simulink model "c00013M_harness"  (R2018a)
settings: Solver=FixedStepAuto  StartTime=0.0  StopTime=300  FixedStep=0.1  RelTol=1e-3
undefined symbols (not defined in the file): A1, hmax, PriorityTank, R1, R2, sigbuilder_block, TempThreshold
(part 1 of 93)
settings Model: Creator=aarrieta  LastModifiedBy=umarkiegi

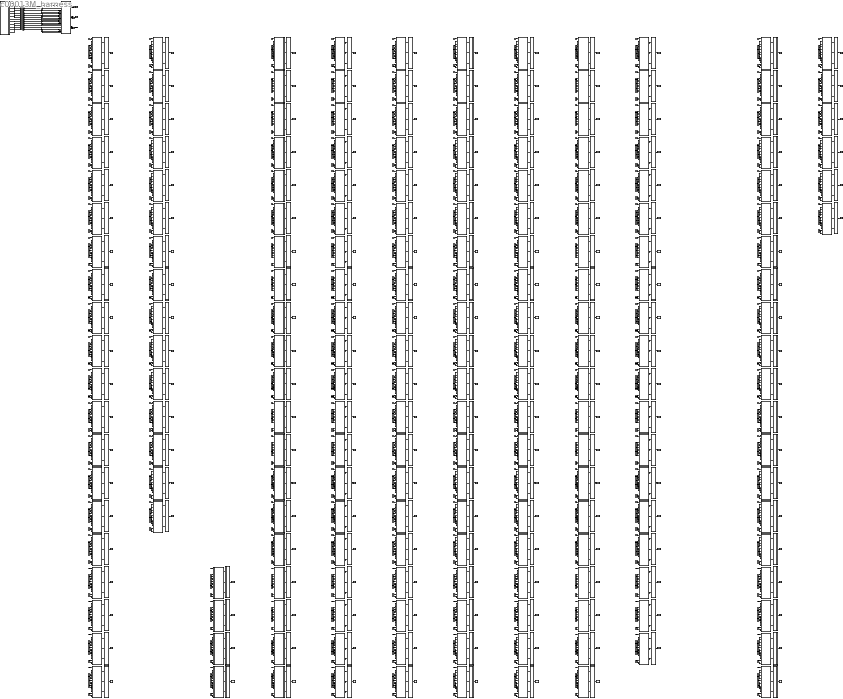
== system c00013M_harness ==
  CPSUT : Subsystem
  Eval : Subsystem
  Eval1 : Subsystem
  Eval10 : Subsystem
  Eval100 : Subsystem
  Eval101 : Subsystem
  Eval102 : Subsystem
  Eval103 : Subsystem
  Eval104 : Subsystem
  Eval105 : Subsystem
  Eval106 : Subsystem
  Eval107 : Subsystem
  Eval108 : Subsystem
  Eval109 : Subsystem
  Eval11 : Subsystem
  Eval110 : Subsystem
  Eval111 : Subsystem
  Eval112 : Subsystem
  Eval113 : Subsystem
  Eval114 : Subsystem
  Eval115 : Subsystem
  Eval116 : Subsystem
  Eval117 : Subsystem
  Eval118 : Subsystem
  Eval119 : Subsystem
  Eval12 : Subsystem
  Eval120 : Subsystem
  Eval121 : Subsystem
  Eval122 : Subsystem
  Eval123 : Subsystem
  Eval124 : Subsystem
  Eval125 : Subsystem
  Eval126 : Subsystem
  Eval127 : Subsystem
  Eval128 : Subsystem
  Eval129 : Subsystem
  Eval13 : Subsystem
  Eval130 : Subsystem
  Eval131 : Subsystem
  Eval132 : Subsystem
  Eval133 : Subsystem
  Eval134 : Subsystem
  Eval135 : Subsystem
  Eval136 : Subsystem
  Eval137 : Subsystem
  Eval138 : Subsystem
  Eval139 : Subsystem
  Eval14 : Subsystem
  Eval140 : Subsystem
  Eval141 : Subsystem
  Eval142 : Subsystem
  Eval143 : Subsystem
  Eval144 : Subsystem
  Eval145 : Subsystem
  Eval146 : Subsystem
  Eval147 : Subsystem
  Eval148 : Subsystem
  Eval149 : Subsystem
  Eval15 : Subsystem
  Eval150 : Subsystem
  Eval151 : Subsystem
  Eval152 : Subsystem
  Eval153 : Subsystem
  Eval154 : Subsystem
  Eval155 : Subsystem
  Eval156 : Subsystem
  Eval157 : Subsystem
  Eval158 : Subsystem
  Eval159 : Subsystem
  Eval16 : Subsystem
  Eval160 : Subsystem
  Eval161 : Subsystem
  Eval162 : Subsystem
  Eval163 : Subsystem
  Eval164 : Subsystem
  Eval165 : Subsystem
  Eval166 : Subsystem
  Eval167 : Subsystem
  Eval168 : Subsystem
  Eval169 : Subsystem
  Eval17 : Subsystem
  Eval170 : Subsystem
  Eval171 : Subsystem
  Eval172 : Subsystem
  Eval173 : Subsystem
  Eval174 : Subsystem
  Eval175 : Subsystem
  Eval176 : Subsystem
  Eval177 : Subsystem
  Eval178 : Subsystem
  Eval179 : Subsystem
  Eval18 : Subsystem
  Eval180 : Subsystem
  Eval181 : Subsystem
  Eval182 : Subsystem
  Eval183 : Subsystem
  Eval184 : Subsystem
  Eval185 : Subsystem
  Eval186 : Subsystem
  Eval187 : Subsystem
  Eval188 : Subsystem
  Eval189 : Subsystem
  Eval19 : Subsystem
  Eval190 : Subsystem
  Eval191 : Subsystem
  Eval192 : Subsystem
  Eval193 : Subsystem
  Eval194 : Subsystem
  Eval195 : Subsystem
  Eval196 : Subsystem
  Eval197 : Subsystem
  Eval198 : Subsystem
  Eval2 : Subsystem
  Eval20 : Subsystem
  Eval21 : Subsystem
  Eval22 : Subsystem
  Eval220 : Subsystem
  Eval221 : Subsystem
  Eval222 : Subsystem
  Eval223 : Subsystem
  Eval224 : Subsystem
  Eval225 : Subsystem
  Eval226 : Subsystem
  Eval227 : Subsystem
  Eval228 : Subsystem
  Eval229 : Subsystem
  Eval23 : Subsystem
  Eval230 : Subsystem
  Eval231 : Subsystem
  Eval232 : Subsystem
  Eval233 : Subsystem
  Eval234 : Subsystem
  Eval235 : Subsystem
  Eval236 : Subsystem
  Eval237 : Subsystem
  Eval238 : Subsystem
  Eval239 : Subsystem
  Eval24 : Subsystem
  Eval240 : Subsystem
  Eval241 : Subsystem
  Eval242 : Subsystem
  Eval243 : Subsystem
  Eval244 : Subsystem
  Eval245 : Subsystem
  Eval25 : Subsystem
  Eval26 : Subsystem
  Eval27 : Subsystem
  Eval28 : Subsystem
  Eval29 : Subsystem
  Eval3 : Subsystem
  Eval30 : Subsystem
  Eval31 : Subsystem
  Eval32 : Subsystem
  Eval33 : Subsystem
  Eval34 : Subsystem
  Eval4 : Subsystem
  Eval5 : Subsystem
  Eval56 : Subsystem
  Eval57 : Subsystem
  Eval58 : Subsystem
  Eval59 : Subsystem
  Eval6 : Subsystem
  Eval60 : Subsystem
  Eval61 : Subsystem
  Eval62 : Subsystem
  Eval63 : Subsystem
  Eval64 : Subsystem
  Eval65 : Subsystem
  Eval66 : Subsystem
  Eval67 : Subsystem
  Eval68 : Subsystem
  Eval69 : Subsystem
  Eval7 : Subsystem
  Eval70 : Subsystem
  Eval71 : Subsystem
  Eval72 : Subsystem
  Eval73 : Subsystem
  Eval74 : Subsystem
  Eval75 : Subsystem
  Eval76 : Subsystem
  Eval77 : Subsystem
  Eval78 : Subsystem
  Eval79 : Subsystem
  Eval8 : Subsystem
  Eval80 : Subsystem
  Eval81 : Subsystem
  Eval82 : Subsystem
  Eval83 : Subsystem
  Eval84 : Subsystem
  Eval85 : Subsystem
  Eval86 : Subsystem
  Eval87 : Subsystem
  Eval88 : Subsystem
  Eval89 : Subsystem
  Eval9 : Subsystem
  Eval90 : Subsystem
  Eval91 : Subsystem
  Eval92 : Subsystem
  Eval93 : Subsystem
  Eval94 : Subsystem
  Eval95 : Subsystem
  Eval96 : Subsystem
  Eval97 : Subsystem
  Eval98 : Subsystem
  Eval99 : Subsystem
  Inputs : Subsystem  Tag=STV Subsys  LoadFcn=sigbuilder_block('load');  StartFcn=sigbuilder_block('start');  StopFcn=sigbuilder_block('stop');  ClipboardFcn=sigbuilder_block('clipboard');  mask(Sigbuilder block){tuvar=[0:10]}
      mask init:
      | if ~strcmp(get_param(bdroot(gcb),'SimulationStatus'),'stopped'),tuvar = sigbuilder_block('maskInit'); end
      settings: CopyFcn=sigbuilder_block('copy');  DeleteFcn=sigbuilder_block('delete');  ModelCloseFcn=sigbuilder_block('modelClose');  PreSaveFcn=sigbuilder_block('preSave');  PauseFcn=sigbuilder_block('pause');  ContinueFcn=sigbuilder_block('continue');  NameChangeFcn=sigbuilder_block('namechange');  OpenFcn=sigbuilder_block('open',[276.75 163.5 675.75 486.75 ]);  CloseFcn=sigbuilder_block('close');
      mask Display: plot(0, 0, 100, 100,[2, 2, 32, 32, 2], [68, 8, 8, 68, 68],[32, 2], [38, 38], [32, 19, 2],[53, 60, 44], [32, 17, 17, 2],[16, 16, 31, 31]);txt = getActiveGroup(gcbh);text(2, 100, txt,'verticalAlignment', 'top');
  M001 : Subsystem
  M002 : Subsystem
  M003 : Subsystem
  M004 : Subsystem
  M005 : Subsystem
  M006 : Subsystem
  M007 : Subsystem
  M008 : Subsystem
  M009 : Subsystem
  M010 : Subsystem
  M011 : Subsystem
  M012 : Subsystem
  M013 : Subsystem
  M014 : Subsystem
  M015 : Subsystem
  M016 : Subsystem
  M017 : Subsystem
  M018 : Subsystem
  M019 : Subsystem
  M020 : Subsystem
  M021 : Subsystem
  M022 : Subsystem
  M023 : Subsystem
  M024 : Subsystem
  M025 : Subsystem
  M026 : Subsystem
  M027 : Subsystem
  M028 : Subsystem
  M029 : Subsystem
  M030 : Subsystem
  M031 : Subsystem
  M032 : Subsystem
  M033 : Subsystem
  M034 : Subsystem
  M035 : Subsystem
  M057 : Subsystem
  M058 : Subsystem
  M059 : Subsystem
  M060 : Subsystem
  M061 : Subsystem
  M062 : Subsystem
  M063 : Subsystem
  M064 : Subsystem
  M065 : Subsystem
  M066 : Subsystem
  M067 : Subsystem
  M068 : Subsystem
  M069 : Subsystem
  M070 : Subsystem
  M071 : Subsystem
  M072 : Subsystem
  M073 : Subsystem
  M074 : Subsystem
  M075 : Subsystem
  M076 : Subsystem
  M077 : Subsystem
  M078 : Subsystem
  M079 : Subsystem
  M080 : Subsystem
  M081 : Subsystem
  M082 : Subsystem
  M083 : Subsystem
  M084 : Subsystem
  M085 : Subsystem
  M086 : Subsystem
  M087 : Subsystem
  M088 : Subsystem
  M089 : Subsystem
  M090 : Subsystem
  M091 : Subsystem
  M092 : Subsystem
  M093 : Subsystem
  M094 : Subsystem
  M095 : Subsystem
  M096 : Subsystem
  M097 : Subsystem
  M098 : Subsystem
  M099 : Subsystem
  M100 : Subsystem
  M101 : Subsystem
  M102 : Subsystem
  M103 : Subsystem
  M104 : Subsystem
  M105 : Subsystem
  M106 : Subsystem
  M107 : Subsystem
  M108 : Subsystem
  M109 : Subsystem
  M110 : Subsystem
  M111 : Subsystem
  M112 : Subsystem
  M113 : Subsystem
  M114 : Subsystem
  M115 : Subsystem
  M116 : Subsystem
  M117 : Subsystem
  M118 : Subsystem
  M119 : Subsystem
  M120 : Subsystem
  M121 : Subsystem
  M122 : Subsystem
  M123 : Subsystem
  M124 : Subsystem
  M125 : Subsystem
  M126 : Subsystem
  M127 : Subsystem
  M128 : Subsystem
  M129 : Subsystem
  M130 : Subsystem
  M131 : Subsystem
  M132 : Subsystem
  M133 : Subsystem
  M134 : Subsystem
  M135 : Subsystem
  M136 : Subsystem
  M137 : Subsystem
  M138 : Subsystem
  M139 : Subsystem
  M140 : Subsystem
  M141 : Subsystem
  M142 : Subsystem
  M143 : Subsystem
  M144 : Subsystem
  M145 : Subsystem
  M146 : Subsystem
  M147 : Subsystem
  M148 : Subsystem
  M149 : Subsystem
  M150 : Subsystem
  M151 : Subsystem
  M152 : Subsystem
  M153 : Subsystem
  M154 : Subsystem
  M155 : Subsystem
  M156 : Subsystem
  M157 : Subsystem
  M158 : Subsystem
  M159 : Subsystem
  M160 : Subsystem
  M161 : Subsystem
  M162 : Subsystem
  M163 : Subsystem
  M164 : Subsystem
  M165 : Subsystem
  M166 : Subsystem
  M167 : Subsystem
  M168 : Subsystem
  M169 : Subsystem
  M170 : Subsystem
  M171 : Subsystem
  M172 : Subsystem
  M173 : Subsystem
  M174 : Subsystem
  M175 : Subsystem
  M176 : Subsystem
  M177 : Subsystem
  M178 : Subsystem
  M179 : Subsystem
  M180 : Subsystem
  M181 : Subsystem
  M182 : Subsystem
  M183 : Subsystem
  M184 : Subsystem
  M185 : Subsystem
  M186 : Subsystem
  M187 : Subsystem
  M188 : Subsystem
  M189 : Subsystem
  M190 : Subsystem
  M191 : Subsystem
  M192 : Subsystem
  M193 : Subsystem
  M194 : Subsystem
  M195 : Subsystem
  M196 : Subsystem
  M197 : Subsystem
  M198 : Subsystem
  M199 : Subsystem
  M221 : Subsystem
  M222 : Subsystem
  M223 : Subsystem
  M224 : Subsystem
  M225 : Subsystem
  M226 : Subsystem
  M227 : Subsystem
  M228 : Subsystem
  M229 : Subsystem
  M230 : Subsystem
  M231 : Subsystem
  M232 : Subsystem
  M233 : Subsystem
  M234 : Subsystem
  M235 : Subsystem
  M236 : Subsystem
  M237 : Subsystem
  M238 : Subsystem
  M239 : Subsystem
  M240 : Subsystem
  M241 : Subsystem
  M242 : Subsystem
  M243 : Subsystem
  M244 : Subsystem
  M245 : Subsystem
  M246 : Subsystem
  To Workspace : ToWorkspace  VariableName=mutant001  SampleTime=-1
  To Workspace1 : ToWorkspace  VariableName=mutant002  SampleTime=-1
  To Workspace10 : ToWorkspace  VariableName=mutant011  SampleTime=-1
  To Workspace100 : ToWorkspace  VariableName=mutant101  SampleTime=-1
  To Workspace101 : ToWorkspace  VariableName=mutant102  SampleTime=-1
  To Workspace102 : ToWorkspace  VariableName=mutant103  SampleTime=-1
  To Workspace103 : ToWorkspace  VariableName=mutant104  SampleTime=-1
  To Workspace104 : ToWorkspace  VariableName=mutant105  SampleTime=-1
  To Workspace105 : ToWorkspace  VariableName=mutant106  SampleTime=-1
  To Workspace106 : ToWorkspace  VariableName=mutant107  SampleTime=-1
  To Workspace107 : ToWorkspace  VariableName=mutant108  SampleTime=-1
  To Workspace108 : ToWorkspace  VariableName=mutant109  SampleTime=-1
  To Workspace109 : ToWorkspace  VariableName=mutant110  SampleTime=-1
  To Workspace11 : ToWorkspace  VariableName=mutant012  SampleTime=-1
  To Workspace110 : ToWorkspace  VariableName=mutant111  SampleTime=-1
  To Workspace111 : ToWorkspace  VariableName=mutant112  SampleTime=-1
  To Workspace112 : ToWorkspace  VariableName=mutant113  SampleTime=-1
  To Workspace113 : ToWorkspace  VariableName=mutant114  SampleTime=-1
  To Workspace114 : ToWorkspace  VariableName=mutant115  SampleTime=-1
  To Workspace115 : ToWorkspace  VariableName=mutant116  SampleTime=-1
  To Workspace116 : ToWorkspace  VariableName=mutant117  SampleTime=-1
  To Workspace117 : ToWorkspace  VariableName=mutant118  SampleTime=-1
  To Workspace118 : ToWorkspace  VariableName=mutant119  SampleTime=-1
  To Workspace119 : ToWorkspace  VariableName=mutant120  SampleTime=-1
  To Workspace12 : ToWorkspace  VariableName=mutant013  SampleTime=-1
  To Workspace120 : ToWorkspace  VariableName=mutant121  SampleTime=-1
  To Workspace121 : ToWorkspace  VariableName=mutant122  SampleTime=-1
  To Workspace122 : ToWorkspace  VariableName=mutant123  SampleTime=-1
  To Workspace123 : ToWorkspace  VariableName=mutant124  SampleTime=-1
  To Workspace124 : ToWorkspace  VariableName=mutant125  SampleTime=-1
  To Workspace125 : ToWorkspace  VariableName=mutant126  SampleTime=-1
  To Workspace126 : ToWorkspace  VariableName=mutant127  SampleTime=-1
  To Workspace127 : ToWorkspace  VariableName=mutant128  SampleTime=-1
  To Workspace128 : ToWorkspace  VariableName=mutant129  SampleTime=-1
  To Workspace129 : ToWorkspace  VariableName=mutant130  SampleTime=-1
  To Workspace13 : ToWorkspace  VariableName=mutant014  SampleTime=-1
  To Workspace130 : ToWorkspace  VariableName=mutant131  SampleTime=-1
  To Workspace131 : ToWorkspace  VariableName=mutant132  SampleTime=-1
  To Workspace132 : ToWorkspace  VariableName=mutant133  SampleTime=-1
  To Workspace133 : ToWorkspace  VariableName=mutant134  SampleTime=-1
  To Workspace134 : ToWorkspace  VariableName=mutant135  SampleTime=-1
  To Workspace135 : ToWorkspace  VariableName=mutant136  SampleTime=-1
  To Workspace136 : ToWorkspace  VariableName=mutant137  SampleTime=-1
  To Workspace137 : ToWorkspace  VariableName=mutant138  SampleTime=-1
  To Workspace138 : ToWorkspace  VariableName=mutant139  SampleTime=-1
  To Workspace139 : ToWorkspace  VariableName=mutant140  SampleTime=-1
  To Workspace14 : ToWorkspace  VariableName=mutant015  SampleTime=-1
  To Workspace140 : ToWorkspace  VariableName=mutant141  SampleTime=-1
  To Workspace141 : ToWorkspace  VariableName=mutant142  SampleTime=-1
  To Workspace142 : ToWorkspace  VariableName=mutant143  SampleTime=-1
  To Workspace143 : ToWorkspace  VariableName=mutant144  SampleTime=-1
  To Workspace144 : ToWorkspace  VariableName=mutant145  SampleTime=-1
  To Workspace145 : ToWorkspace  VariableName=mutant146  SampleTime=-1
  To Workspace146 : ToWorkspace  VariableName=mutant147  SampleTime=-1
  To Workspace147 : ToWorkspace  VariableName=mutant148  SampleTime=-1
  To Workspace148 : ToWorkspace  VariableName=mutant149  SampleTime=-1
  To Workspace149 : ToWorkspace  VariableName=mutant150  SampleTime=-1
  To Workspace15 : ToWorkspace  VariableName=mutant016  SampleTime=-1
  To Workspace150 : ToWorkspace  VariableName=mutant151  SampleTime=-1
  To Workspace151 : ToWorkspace  VariableName=mutant152  SampleTime=-1
  To Workspace152 : ToWorkspace  VariableName=mutant153  SampleTime=-1
  To Workspace153 : ToWorkspace  VariableName=mutant154  SampleTime=-1
  To Workspace154 : ToWorkspace  VariableName=mutant155  SampleTime=-1
  To Workspace155 : ToWorkspace  VariableName=mutant156  SampleTime=-1
  To Workspace156 : ToWorkspace  VariableName=mutant157  SampleTime=-1
  To Workspace157 : ToWorkspace  VariableName=mutant158  SampleTime=-1
  To Workspace158 : ToWorkspace  VariableName=mutant159  SampleTime=-1
  To Workspace159 : ToWorkspace  VariableName=mutant160  SampleTime=-1
  To Workspace16 : ToWorkspace  VariableName=mutant017  SampleTime=-1
  To Workspace160 : ToWorkspace  VariableName=mutant161  SampleTime=-1
  To Workspace161 : ToWorkspace  VariableName=mutant162  SampleTime=-1
  To Workspace162 : ToWorkspace  VariableName=mutant163  SampleTime=-1
  To Workspace163 : ToWorkspace  VariableName=mutant164  SampleTime=-1
  To Workspace164 : ToWorkspace  VariableName=mutant165  SampleTime=-1
  To Workspace165 : ToWorkspace  VariableName=mutant166  SampleTime=-1
  To Workspace166 : ToWorkspace  VariableName=mutant167  SampleTime=-1
  To Workspace167 : ToWorkspace  VariableName=mutant168  SampleTime=-1
  To Workspace168 : ToWorkspace  VariableName=mutant169  SampleTime=-1
  To Workspace169 : ToWorkspace  VariableName=mutant170  SampleTime=-1
  To Workspace17 : ToWorkspace  VariableName=mutant018  SampleTime=-1
  To Workspace170 : ToWorkspace  VariableName=mutant171  SampleTime=-1
  To Workspace171 : ToWorkspace  VariableName=mutant172  SampleTime=-1
  To Workspace172 : ToWorkspace  VariableName=mutant173  SampleTime=-1
  To Workspace173 : ToWorkspace  VariableName=mutant174  SampleTime=-1
  To Workspace174 : ToWorkspace  VariableName=mutant175  SampleTime=-1
  To Workspace175 : ToWorkspace  VariableName=mutant176  SampleTime=-1
  To Workspace176 : ToWorkspace  VariableName=mutant177  SampleTime=-1
  To Workspace177 : ToWorkspace  VariableName=mutant178  SampleTime=-1
  To Workspace178 : ToWorkspace  VariableName=mutant179  SampleTime=-1
  To Workspace179 : ToWorkspace  VariableName=mutant180  SampleTime=-1
  To Workspace18 : ToWorkspace  VariableName=mutant019  SampleTime=-1
  To Workspace180 : ToWorkspace  VariableName=mutant181  SampleTime=-1
  To Workspace181 : ToWorkspace  VariableName=mutant182  SampleTime=-1
  To Workspace182 : ToWorkspace  VariableName=mutant183  SampleTime=-1
  To Workspace183 : ToWorkspace  VariableName=mutant184  SampleTime=-1
  To Workspace184 : ToWorkspace  VariableName=mutant185  SampleTime=-1
  To Workspace185 : ToWorkspace  VariableName=mutant186  SampleTime=-1
  To Workspace186 : ToWorkspace  VariableName=mutant187  SampleTime=-1
  To Workspace187 : ToWorkspace  VariableName=mutant188  SampleTime=-1
  To Workspace188 : ToWorkspace  VariableName=mutant189  SampleTime=-1
  To Workspace189 : ToWorkspace  VariableName=mutant190  SampleTime=-1
  To Workspace19 : ToWorkspace  VariableName=mutant020  SampleTime=-1
  To Workspace190 : ToWorkspace  VariableName=mutant191  SampleTime=-1
  To Workspace191 : ToWorkspace  VariableName=mutant192  SampleTime=-1
  To Workspace192 : ToWorkspace  VariableName=mutant193  SampleTime=-1
  To Workspace193 : ToWorkspace  VariableName=mutant194  SampleTime=-1
  To Workspace194 : ToWorkspace  VariableName=mutant195  SampleTime=-1
  To Workspace195 : ToWorkspace  VariableName=mutant196  SampleTime=-1
  To Workspace196 : ToWorkspace  VariableName=mutant197  SampleTime=-1
  To Workspace197 : ToWorkspace  VariableName=mutant198  SampleTime=-1
  To Workspace198 : ToWorkspace  VariableName=mutant199  SampleTime=-1
  To Workspace2 : ToWorkspace  VariableName=mutant003  SampleTime=-1
  To Workspace20 : ToWorkspace  VariableName=mutant021  SampleTime=-1
  To Workspace21 : ToWorkspace  VariableName=mutant022  SampleTime=-1
  To Workspace22 : ToWorkspace  VariableName=mutant023  SampleTime=-1
  To Workspace220 : ToWorkspace  VariableName=mutant221  SampleTime=-1
  To Workspace221 : ToWorkspace  VariableName=mutant222  SampleTime=-1
  To Workspace222 : ToWorkspace  VariableName=mutant223  SampleTime=-1
  To Workspace223 : ToWorkspace  VariableName=mutant224  SampleTime=-1
  To Workspace224 : ToWorkspace  VariableName=mutant225  SampleTime=-1
  To Workspace225 : ToWorkspace  VariableName=mutant226  SampleTime=-1
  To Workspace226 : ToWorkspace  VariableName=mutant227  SampleTime=-1
  To Workspace227 : ToWorkspace  VariableName=mutant228  SampleTime=-1
  To Workspace228 : ToWorkspace  VariableName=mutant229  SampleTime=-1
  To Workspace229 : ToWorkspace  VariableName=mutant230  SampleTime=-1
  To Workspace23 : ToWorkspace  VariableName=mutant024  SampleTime=-1
  To Workspace230 : ToWorkspace  VariableName=mutant231  SampleTime=-1
  To Workspace231 : ToWorkspace  VariableName=mutant232  SampleTime=-1
  To Workspace232 : ToWorkspace  VariableName=mutant233  SampleTime=-1
  To Workspace233 : ToWorkspace  VariableName=mutant234  SampleTime=-1
  To Workspace234 : ToWorkspace  VariableName=mutant235  SampleTime=-1
  To Workspace235 : ToWorkspace  VariableName=mutant236  SampleTime=-1
  To Workspace236 : ToWorkspace  VariableName=mutant237  SampleTime=-1
  To Workspace237 : ToWorkspace  VariableName=mutant238  SampleTime=-1
  To Workspace238 : ToWorkspace  VariableName=mutant239  SampleTime=-1
  To Workspace239 : ToWorkspace  VariableName=mutant240  SampleTime=-1
  To Workspace24 : ToWorkspace  VariableName=mutant025  SampleTime=-1
  To Workspace240 : ToWorkspace  VariableName=mutant241  SampleTime=-1
  To Workspace241 : ToWorkspace  VariableName=mutant242  SampleTime=-1
  To Workspace242 : ToWorkspace  VariableName=mutant243  SampleTime=-1
  To Workspace243 : ToWorkspace  VariableName=mutant244  SampleTime=-1
  To Workspace244 : ToWorkspace  VariableName=mutant245  SampleTime=-1
  To Workspace245 : ToWorkspace  VariableName=mutant246  SampleTime=-1
  To Workspace25 : ToWorkspace  VariableName=mutant026  SampleTime=-1
  To Workspace26 : ToWorkspace  VariableName=mutant027  SampleTime=-1
  To Workspace27 : ToWorkspace  VariableName=mutant028  SampleTime=-1
  To Workspace28 : ToWorkspace  VariableName=mutant029  SampleTime=-1
  To Workspace29 : ToWorkspace  VariableName=mutant030  SampleTime=-1
  To Workspace3 : ToWorkspace  VariableName=mutant004  SampleTime=-1
  To Workspace30 : ToWorkspace  VariableName=mutant031  SampleTime=-1
  To Workspace31 : ToWorkspace  VariableName=mutant032  SampleTime=-1
  To Workspace32 : ToWorkspace  VariableName=mutant033  SampleTime=-1
  To Workspace33 : ToWorkspace  VariableName=mutant034  SampleTime=-1
  To Workspace34 : ToWorkspace  VariableName=mutant035  SampleTime=-1
  To Workspace4 : ToWorkspace  VariableName=mutant005  SampleTime=-1
  To Workspace5 : ToWorkspace  VariableName=mutant006  SampleTime=-1
  To Workspace56 : ToWorkspace  VariableName=mutant057  SampleTime=-1
  To Workspace57 : ToWorkspace  VariableName=mutant058  SampleTime=-1
  To Workspace58 : ToWorkspace  VariableName=mutant059  SampleTime=-1
  To Workspace59 : ToWorkspace  VariableName=mutant060  SampleTime=-1
  To Workspace6 : ToWorkspace  VariableName=mutant007  SampleTime=-1
  To Workspace60 : ToWorkspace  VariableName=mutant061  SampleTime=-1
  To Workspace61 : ToWorkspace  VariableName=mutant062  SampleTime=-1
  To Workspace62 : ToWorkspace  VariableName=mutant063  SampleTime=-1
  To Workspace63 : ToWorkspace  VariableName=mutant064  SampleTime=-1
  To Workspace64 : ToWorkspace  VariableName=mutant065  SampleTime=-1
  To Workspace65 : ToWorkspace  VariableName=mutant066  SampleTime=-1
  To Workspace66 : ToWorkspace  VariableName=mutant067  SampleTime=-1
  To Workspace67 : ToWorkspace  VariableName=mutant068  SampleTime=-1
  To Workspace68 : ToWorkspace  VariableName=mutant069  SampleTime=-1
  To Workspace69 : ToWorkspace  VariableName=mutant070  SampleTime=-1
  To Workspace7 : ToWorkspace  VariableName=mutant008  SampleTime=-1
  To Workspace70 : ToWorkspace  VariableName=mutant071  SampleTime=-1
  To Workspace71 : ToWorkspace  VariableName=mutant072  SampleTime=-1
  To Workspace72 : ToWorkspace  VariableName=mutant073  SampleTime=-1
  To Workspace73 : ToWorkspace  VariableName=mutant074  SampleTime=-1
  To Workspace74 : ToWorkspace  VariableName=mutant075  SampleTime=-1
  To Workspace75 : ToWorkspace  VariableName=mutant076  SampleTime=-1
  To Workspace76 : ToWorkspace  VariableName=mutant077  SampleTime=-1
  To Workspace77 : ToWorkspace  VariableName=mutant078  SampleTime=-1
  To Workspace78 : ToWorkspace  VariableName=mutant079  SampleTime=-1
  To Workspace79 : ToWorkspace  VariableName=mutant080  SampleTime=-1
  To Workspace8 : ToWorkspace  VariableName=mutant009  SampleTime=-1
  To Workspace80 : ToWorkspace  VariableName=mutant081  SampleTime=-1
  To Workspace81 : ToWorkspace  VariableName=mutant082  SampleTime=-1
  To Workspace82 : ToWorkspace  VariableName=mutant083  SampleTime=-1
  To Workspace83 : ToWorkspace  VariableName=mutant084  SampleTime=-1
  To Workspace84 : ToWorkspace  VariableName=mutant085  SampleTime=-1
  To Workspace85 : ToWorkspace  VariableName=mutant086  SampleTime=-1
  To Workspace86 : ToWorkspace  VariableName=mutant087  SampleTime=-1
  To Workspace87 : ToWorkspace  VariableName=mutant088  SampleTime=-1
  To Workspace88 : ToWorkspace  VariableName=mutant089  SampleTime=-1
  To Workspace89 : ToWorkspace  VariableName=mutant090  SampleTime=-1
  To Workspace9 : ToWorkspace  VariableName=mutant010  SampleTime=-1
  To Workspace90 : ToWorkspace  VariableName=mutant091  SampleTime=-1
  To Workspace91 : ToWorkspace  VariableName=mutant092  SampleTime=-1
  To Workspace92 : ToWorkspace  VariableName=mutant093  SampleTime=-1
  To Workspace93 : ToWorkspace  VariableName=mutant094  SampleTime=-1
  To Workspace94 : ToWorkspace  VariableName=mutant095  SampleTime=-1
  To Workspace95 : ToWorkspace  VariableName=mutant096  SampleTime=-1
  To Workspace96 : ToWorkspace  VariableName=mutant097  SampleTime=-1
  To Workspace97 : ToWorkspace  VariableName=mutant098  SampleTime=-1
  To Workspace98 : ToWorkspace  VariableName=mutant099  SampleTime=-1
  To Workspace99 : ToWorkspace  VariableName=mutant100  SampleTime=-1
  dtc_CT1 : DataTypeConversion
  dtc_CT2 : DataTypeConversion
  dtc_CT3 : DataTypeConversion
  dtc_E2 : DataTypeConversion
  dtc_EB1 : DataTypeConversion
  dtc_EB2 : DataTypeConversion
  dtc_EB3 : DataTypeConversion
  dtc_F2 : DataTypeConversion
  dtc_MR2 : DataTypeConversion
  dtc_T1 : DataTypeConversion
  dtc_T2 : DataTypeConversion
  dtc_T3 : DataTypeConversion
  LL1 : Outport
  LL2 : Outport  Port=2
  LL3 : Outport  Port=3
  tag scope: out1=global, out2=global, out3=global
  wires:
  CPSUT/1(LL1) -> [out1], LL1/1
  CPSUT/2(LL2) -> [out2], LL2/1
  CPSUT/3(LL3) -> [out3], LL3/1
  [in1] -> M001/1(CT1)
  [in5] -> M001/2(T1)
  [in6] -> M001/3(EB1)
  [in7] -> M001/4(CT2)
  [in8] -> M001/5(F2)
  [in9] -> M001/6(E2)
  [in10] -> M001/7(MR2)
  [in11] -> M001/8(T2)
  [in12] -> M001/9(EB2)
  [in13] -> M001/10(CT3)
  [in17] -> M001/11(T3)
  [in18] -> M001/12(EB3)
  Eval/1(Out1) -> To Workspace/1
  M001/1(LL1) -> Eval/1(In1)
  M001/2(LL2) -> Eval/2(In2)
  M001/3(LL3) -> Eval/3(In3)
  [in1] -> M002/1(CT1)
  [in5] -> M002/2(T1)
  [in6] -> M002/3(EB1)
  [in7] -> M002/4(CT2)
  [in8] -> M002/5(F2)
  [in9] -> M002/6(E2)
  [in10] -> M002/7(MR2)
  [in11] -> M002/8(T2)
  [in12] -> M002/9(EB2)
  [in13] -> M002/10(CT3)
  [in17] -> M002/11(T3)
  [in18] -> M002/12(EB3)
  M002/1(LL1) -> Eval1/1(In1)
  M002/2(LL2) -> Eval1/2(In2)
  M002/3(LL3) -> Eval1/3(In3)
  Eval1/1(Out1) -> To Workspace1/1
  [in1] -> M003/1(CT1)
  [in5] -> M003/2(T1)
  [in6] -> M003/3(EB1)
  [in7] -> M003/4(CT2)
  [in8] -> M003/5(F2)
  [in9] -> M003/6(E2)
  [in10] -> M003/7(MR2)
  [in11] -> M003/8(T2)
  [in12] -> M003/9(EB2)
  [in13] -> M003/10(CT3)
  [in17] -> M003/11(T3)
  [in18] -> M003/12(EB3)
  M003/1(LL1) -> Eval2/1(In1)
  M003/2(LL2) -> Eval2/2(In2)
  M003/3(LL3) -> Eval2/3(In3)
  Eval2/1(Out1) -> To Workspace2/1
  [in1] -> M004/1(CT1)
  [in5] -> M004/2(T1)
  [in6] -> M004/3(EB1)
  [in7] -> M004/4(CT2)
  [in8] -> M004/5(F2)
  [in9] -> M004/6(E2)
  [in10] -> M004/7(MR2)
  [in11] -> M004/8(T2)
  [in12] -> M004/9(EB2)
  [in13] -> M004/10(CT3)
  [in17] -> M004/11(T3)
  [in18] -> M004/12(EB3)
  M004/1(LL1) -> Eval3/1(In1)
  M004/2(LL2) -> Eval3/2(In2)
  M004/3(LL3) -> Eval3/3(In3)
  Eval3/1(Out1) -> To Workspace3/1
  [in1] -> M005/1(CT1)
  [in5] -> M005/2(T1)
  [in6] -> M005/3(EB1)
  [in7] -> M005/4(CT2)
  [in8] -> M005/5(F2)
  [in9] -> M005/6(E2)
  [in10] -> M005/7(MR2)
  [in11] -> M005/8(T2)
  [in12] -> M005/9(EB2)
  [in13] -> M005/10(CT3)
  [in17] -> M005/11(T3)
  [in18] -> M005/12(EB3)
  M005/1(LL1) -> Eval4/1(In1)
  M005/2(LL2) -> Eval4/2(In2)
  M005/3(LL3) -> Eval4/3(In3)
  Eval4/1(Out1) -> To Workspace4/1
  [in1] -> M006/1(CT1)
  [in5] -> M006/2(T1)
  [in6] -> M006/3(EB1)
  [in7] -> M006/4(CT2)
  [in8] -> M006/5(F2)
  [in9] -> M006/6(E2)
  [in10] -> M006/7(MR2)
  [in11] -> M006/8(T2)
  [in12] -> M006/9(EB2)
  [in13] -> M006/10(CT3)
  [in17] -> M006/11(T3)
  [in18] -> M006/12(EB3)
  M006/1(LL1) -> Eval5/1(In1)
  M006/2(LL2) -> Eval5/2(In2)
  M006/3(LL3) -> Eval5/3(In3)
  Eval5/1(Out1) -> To Workspace5/1
  [in1] -> M007/1(CT1)
  [in5] -> M007/2(T1)
  [in6] -> M007/3(EB1)
  [in7] -> M007/4(CT2)
  [in8] -> M007/5(F2)
  [in9] -> M007/6(E2)
  [in10] -> M007/7(MR2)
  [in11] -> M007/8(T2)
  [in12] -> M007/9(EB2)
  [in13] -> M007/10(CT3)
  [in17] -> M007/11(T3)
  [in18] -> M007/12(EB3)
  M007/1(LL1) -> Eval6/1(In1)
  M007/2(LL2) -> Eval6/2(In2)
  M007/3(LL3) -> Eval6/3(In3)
  Eval6/1(Out1) -> To Workspace6/1
  [in1] -> M008/1(CT1)
  [in5] -> M008/2(T1)
  [in6] -> M008/3(EB1)
  [in7] -> M008/4(CT2)
  [in8] -> M008/5(F2)
  [in9] -> M008/6(E2)
  [in10] -> M008/7(MR2)
  [in11] -> M008/8(T2)
  [in12] -> M008/9(EB2)
  [in13] -> M008/10(CT3)
  [in17] -> M008/11(T3)
  [in18] -> M008/12(EB3)
  M008/1(LL1) -> Eval7/1(In1)
  M008/2(LL2) -> Eval7/2(In2)
  M008/3(LL3) -> Eval7/3(In3)
  Eval7/1(Out1) -> To Workspace7/1
  [in1] -> M009/1(CT1)
  [in5] -> M009/2(T1)
  [in6] -> M009/3(EB1)
  [in7] -> M009/4(CT2)
  [in8] -> M009/5(F2)
  [in9] -> M009/6(E2)
  [in10] -> M009/7(MR2)
  [in11] -> M009/8(T2)
  [in12] -> M009/9(EB2)
  [in13] -> M009/10(CT3)
  [in17] -> M009/11(T3)
  [in18] -> M009/12(EB3)
  M009/1(LL1) -> Eval8/1(In1)
  M009/2(LL2) -> Eval8/2(In2)
  M009/3(LL3) -> Eval8/3(In3)
  Eval8/1(Out1) -> To Workspace8/1
  [in1] -> M010/1(CT1)
  [in5] -> M010/2(T1)
  [in6] -> M010/3(EB1)
  [in7] -> M010/4(CT2)
  [in8] -> M010/5(F2)
  [in9] -> M010/6(E2)
  [in10] -> M010/7(MR2)
  [in11] -> M010/8(T2)
  [in12] -> M010/9(EB2)
  [in13] -> M010/10(CT3)
  [in17] -> M010/11(T3)
  [in18] -> M010/12(EB3)
  M010/1(LL1) -> Eval9/1(In1)
  M010/2(LL2) -> Eval9/2(In2)
  M010/3(LL3) -> Eval9/3(In3)
  Eval9/1(Out1) -> To Workspace9/1
  [in1] -> M011/1(CT1)
  [in5] -> M011/2(T1)
  [in6] -> M011/3(EB1)
  [in7] -> M011/4(CT2)
  [in8] -> M011/5(F2)
  [in9] -> M011/6(E2)
  [in10] -> M011/7(MR2)
  [in11] -> M011/8(T2)
  [in12] -> M011/9(EB2)
  [in13] -> M011/10(CT3)
  [in17] -> M011/11(T3)
  [in18] -> M011/12(EB3)
  M011/1(LL1) -> Eval10/1(In1)
  M011/2(LL2) -> Eval10/2(In2)
  M011/3(LL3) -> Eval10/3(In3)
  Eval10/1(Out1) -> To Workspace10/1
  [in1] -> M012/1(CT1)
  [in5] -> M012/2(T1)
  [in6] -> M012/3(EB1)
  [in7] -> M012/4(CT2)
  [in8] -> M012/5(F2)
  [in9] -> M012/6(E2)
  [in10] -> M012/7(MR2)
  [in11] -> M012/8(T2)
  [in12] -> M012/9(EB2)
  [in13] -> M012/10(CT3)
  [in17] -> M012/11(T3)
  [in18] -> M012/12(EB3)
  M012/1(LL1) -> Eval11/1(In1)
  M012/2(LL2) -> Eval11/2(In2)
  M012/3(LL3) -> Eval11/3(In3)
  Eval11/1(Out1) -> To Workspace11/1
  [in1] -> M013/1(CT1)
  [in5] -> M013/2(T1)
  [in6] -> M013/3(EB1)
  [in7] -> M013/4(CT2)
  [in8] -> M013/5(F2)
  [in9] -> M013/6(E2)
  [in10] -> M013/7(MR2)
  [in11] -> M013/8(T2)
  [in12] -> M013/9(EB2)
  [in13] -> M013/10(CT3)
  [in17] -> M013/11(T3)
  [in18] -> M013/12(EB3)
  M013/1(LL1) -> Eval12/1(In1)
  M013/2(LL2) -> Eval12/2(In2)
  M013/3(LL3) -> Eval12/3(In3)
  Eval12/1(Out1) -> To Workspace12/1
  [in1] -> M014/1(CT1)
  [in5] -> M014/2(T1)
  [in6] -> M014/3(EB1)
  [in7] -> M014/4(CT2)
  [in8] -> M014/5(F2)
  [in9] -> M014/6(E2)
  [in10] -> M014/7(MR2)
  [in11] -> M014/8(T2)
  [in12] -> M014/9(EB2)
  [in13] -> M014/10(CT3)
  [in17] -> M014/11(T3)
  [in18] -> M014/12(EB3)
  M014/1(LL1) -> Eval13/1(In1)
  M014/2(LL2) -> Eval13/2(In2)
  M014/3(LL3) -> Eval13/3(In3)
  Eval13/1(Out1) -> To Workspace13/1
  [in1] -> M015/1(CT1)
  [in5] -> M015/2(T1)
  [in6] -> M015/3(EB1)
  [in7] -> M015/4(CT2)
  [in8] -> M015/5(F2)
  [in9] -> M015/6(E2)
  [in10] -> M015/7(MR2)
  [in11] -> M015/8(T2)
  [in12] -> M015/9(EB2)
  [in13] -> M015/10(CT3)
  [in17] -> M015/11(T3)
  [in18] -> M015/12(EB3)
  M015/1(LL1) -> Eval14/1(In1)
  M015/2(LL2) -> Eval14/2(In2)
  M015/3(LL3) -> Eval14/3(In3)
  Eval14/1(Out1) -> To Workspace14/1
  [in1] -> M016/1(CT1)
  [in5] -> M016/2(T1)
  [in6] -> M016/3(EB1)
  [in7] -> M016/4(CT2)
  [in8] -> M016/5(F2)
  [in9] -> M016/6(E2)
  [in10] -> M016/7(MR2)
  [in11] -> M016/8(T2)
  [in12] -> M016/9(EB2)
  [in13] -> M016/10(CT3)
  [in17] -> M016/11(T3)
  [in18] -> M016/12(EB3)
  M016/1(LL1) -> Eval15/1(In1)
  M016/2(LL2) -> Eval15/2(In2)
  M016/3(LL3) -> Eval15/3(In3)
  Eval15/1(Out1) -> To Workspace15/1
  [in1] -> M017/1(CT1)
  [in5] -> M017/2(T1)
  [in6] -> M017/3(EB1)
  [in7] -> M017/4(CT2)
  [in8] -> M017/5(F2)
  [in9] -> M017/6(E2)
  [in10] -> M017/7(MR2)
  [in11] -> M017/8(T2)
  [in12] -> M017/9(EB2)
  [in13] -> M017/10(CT3)
  [in17] -> M017/11(T3)
  [in18] -> M017/12(EB3)
  M017/1(LL1) -> Eval16/1(In1)
  M017/2(LL2) -> Eval16/2(In2)
  M017/3(LL3) -> Eval16/3(In3)
  Eval16/1(Out1) -> To Workspace16/1
  [in1] -> M018/1(CT1)
  [in5] -> M018/2(T1)
  [in6] -> M018/3(EB1)
  [in7] -> M018/4(CT2)
  [in8] -> M018/5(F2)
  [in9] -> M018/6(E2)
  [in10] -> M018/7(MR2)
  [in11] -> M018/8(T2)
  [in12] -> M018/9(EB2)
  [in13] -> M018/10(CT3)
  [in17] -> M018/11(T3)
  [in18] -> M018/12(EB3)
  M018/1(LL1) -> Eval17/1(In1)
  M018/2(LL2) -> Eval17/2(In2)
  M018/3(LL3) -> Eval17/3(In3)
  Eval17/1(Out1) -> To Workspace17/1
  [in1] -> M019/1(CT1)
  [in5] -> M019/2(T1)
  [in6] -> M019/3(EB1)
  [in7] -> M019/4(CT2)
  [in8] -> M019/5(F2)
  [in9] -> M019/6(E2)
  [in10] -> M019/7(MR2)
  [in11] -> M019/8(T2)
  [in12] -> M019/9(EB2)
  [in13] -> M019/10(CT3)
  [in17] -> M019/11(T3)
  [in18] -> M019/12(EB3)
  M019/1(LL1) -> Eval18/1(In1)
  M019/2(LL2) -> Eval18/2(In2)
  M019/3(LL3) -> Eval18/3(In3)
  Eval18/1(Out1) -> To Workspace18/1
  [in1] -> M020/1(CT1)
  [in5] -> M020/2(T1)
  [in6] -> M020/3(EB1)
  [in7] -> M020/4(CT2)
  [in8] -> M020/5(F2)
  [in9] -> M020/6(E2)
  [in10] -> M020/7(MR2)
  [in11] -> M020/8(T2)
  [in12] -> M020/9(EB2)
  [in13] -> M020/10(CT3)
  [in17] -> M020/11(T3)
  [in18] -> M020/12(EB3)
  M020/1(LL1) -> Eval19/1(In1)
  M020/2(LL2) -> Eval19/2(In2)
  M020/3(LL3) -> Eval19/3(In3)
  Eval19/1(Out1) -> To Workspace19/1
  [in1] -> M021/1(CT1)
  [in5] -> M021/2(T1)
  [in6] -> M021/3(EB1)
  [in7] -> M021/4(CT2)
  [in8] -> M021/5(F2)
  [in9] -> M021/6(E2)
  [in10] -> M021/7(MR2)
  [in11] -> M021/8(T2)
  [in12] -> M021/9(EB2)
  [in13] -> M021/10(CT3)
  [in17] -> M021/11(T3)
  [in18] -> M021/12(EB3)
  M021/1(LL1) -> Eval20/1(In1)
  M021/2(LL2) -> Eval20/2(In2)
  M021/3(LL3) -> Eval20/3(In3)
  Eval20/1(Out1) -> To Workspace20/1
  [in1] -> M022/1(CT1)
  [in5] -> M022/2(T1)
  [in6] -> M022/3(EB1)
  [in7] -> M022/4(CT2)
  [in8] -> M022/5(F2)
  [in9] -> M022/6(E2)
  [in10] -> M022/7(MR2)
  [in11] -> M022/8(T2)
  [in12] -> M022/9(EB2)
  [in13] -> M022/10(CT3)
  [in17] -> M022/11(T3)
  [in18] -> M022/12(EB3)
  M022/1(LL1) -> Eval21/1(In1)
  M022/2(LL2) -> Eval21/2(In2)
  M022/3(LL3) -> Eval21/3(In3)
  Eval21/1(Out1) -> To Workspace21/1
  [in1] -> M023/1(CT1)
  [in5] -> M023/2(T1)
  [in6] -> M023/3(EB1)
  [in7] -> M023/4(CT2)
  [in8] -> M023/5(F2)
  [in9] -> M023/6(E2)
  [in10] -> M023/7(MR2)
  [in11] -> M023/8(T2)
  [in12] -> M023/9(EB2)
  [in13] -> M023/10(CT3)
  [in17] -> M023/11(T3)
  [in18] -> M023/12(EB3)
  M023/1(LL1) -> Eval22/1(In1)
  M023/2(LL2) -> Eval22/2(In2)
  M023/3(LL3) -> Eval22/3(In3)
  Eval22/1(Out1) -> To Workspace22/1
  [in1] -> M024/1(CT1)
  [in5] -> M024/2(T1)
  [in6] -> M024/3(EB1)
  [in7] -> M024/4(CT2)
  [in8] -> M024/5(F2)
  [in9] -> M024/6(E2)
  [in10] -> M024/7(MR2)
  [in11] -> M024/8(T2)
  [in12] -> M024/9(EB2)
  [in13] -> M024/10(CT3)
  [in17] -> M024/11(T3)
  [in18] -> M024/12(EB3)
  M024/1(LL1) -> Eval23/1(In1)
  M024/2(LL2) -> Eval23/2(In2)
  M024/3(LL3) -> Eval23/3(In3)
  Eval23/1(Out1) -> To Workspace23/1
  [in1] -> M025/1(CT1)
  [in5] -> M025/2(T1)
  [in6] -> M025/3(EB1)
  [in7] -> M025/4(CT2)
  [in8] -> M025/5(F2)
  [in9] -> M025/6(E2)
  [in10] -> M025/7(MR2)
  [in11] -> M025/8(T2)
  [in12] -> M025/9(EB2)
  [in13] -> M025/10(CT3)
  [in17] -> M025/11(T3)
  [in18] -> M025/12(EB3)
  M025/1(LL1) -> Eval24/1(In1)
  M025/2(LL2) -> Eval24/2(In2)
  M025/3(LL3) -> Eval24/3(In3)
  Eval24/1(Out1) -> To Workspace24/1
  [in1] -> M026/1(CT1)
  [in5] -> M026/2(T1)
  [in6] -> M026/3(EB1)
  [in7] -> M026/4(CT2)
  [in8] -> M026/5(F2)
  [in9] -> M026/6(E2)
  [in10] -> M026/7(MR2)
  [in11] -> M026/8(T2)
  [in12] -> M026/9(EB2)
  [in13] -> M026/10(CT3)
  [in17] -> M026/11(T3)
  [in18] -> M026/12(EB3)
  M026/1(LL1) -> Eval25/1(In1)
  M026/2(LL2) -> Eval25/2(In2)
  M026/3(LL3) -> Eval25/3(In3)
  Eval25/1(Out1) -> To Workspace25/1
  [in1] -> M027/1(CT1)
  [in5] -> M027/2(T1)
  [in6] -> M027/3(EB1)
  [in7] -> M027/4(CT2)
  [in8] -> M027/5(F2)
  [in9] -> M027/6(E2)
  [in10] -> M027/7(MR2)
  [in11] -> M027/8(T2)
  [in12] -> M027/9(EB2)
  [in13] -> M027/10(CT3)
  [in17] -> M027/11(T3)
  [in18] -> M027/12(EB3)
  M027/1(LL1) -> Eval26/1(In1)
  M027/2(LL2) -> Eval26/2(In2)
  M027/3(LL3) -> Eval26/3(In3)
  Eval26/1(Out1) -> To Workspace26/1
  [in1] -> M028/1(CT1)
  [in5] -> M028/2(T1)
  [in6] -> M028/3(EB1)
  [in7] -> M028/4(CT2)
  [in8] -> M028/5(F2)
  [in9] -> M028/6(E2)
  [in10] -> M028/7(MR2)
  [in11] -> M028/8(T2)
  [in12] -> M028/9(EB2)
  [in13] -> M028/10(CT3)
  [in17] -> M028/11(T3)
  [in18] -> M028/12(EB3)
  M028/1(LL1) -> Eval27/1(In1)
  M028/2(LL2) -> Eval27/2(In2)
  M028/3(LL3) -> Eval27/3(In3)
  Eval27/1(Out1) -> To Workspace27/1
  [in1] -> M029/1(CT1)
  [in5] -> M029/2(T1)
  [in6] -> M029/3(EB1)
  [in7] -> M029/4(CT2)
  [in8] -> M029/5(F2)
  [in9] -> M029/6(E2)
  [in10] -> M029/7(MR2)
  [in11] -> M029/8(T2)
  [in12] -> M029/9(EB2)
  [in13] -> M029/10(CT3)
  [in17] -> M029/11(T3)
  [in18] -> M029/12(EB3)
  M029/1(LL1) -> Eval28/1(In1)
  M029/2(LL2) -> Eval28/2(In2)
  M029/3(LL3) -> Eval28/3(In3)
  Eval28/1(Out1) -> To Workspace28/1
  [in1] -> M030/1(CT1)
  [in5] -> M030/2(T1)
  [in6] -> M030/3(EB1)
  [in7] -> M030/4(CT2)
  [in8] -> M030/5(F2)
  [in9] -> M030/6(E2)
  [in10] -> M030/7(MR2)
  [in11] -> M030/8(T2)
  [in12] -> M030/9(EB2)
  [in13] -> M030/10(CT3)
  [in17] -> M030/11(T3)
  [in18] -> M030/12(EB3)
  M030/1(LL1) -> Eval29/1(In1)
  M030/2(LL2) -> Eval29/2(In2)
  M030/3(LL3) -> Eval29/3(In3)
  Eval29/1(Out1) -> To Workspace29/1
  [in1] -> M031/1(CT1)
  [in5] -> M031/2(T1)
  [in6] -> M031/3(EB1)
  [in7] -> M031/4(CT2)
  [in8] -> M031/5(F2)
  [in9] -> M031/6(E2)
  [in10] -> M031/7(MR2)
  [in11] -> M031/8(T2)
  [in12] -> M031/9(EB2)
  [in13] -> M031/10(CT3)
  [in17] -> M031/11(T3)
  [in18] -> M031/12(EB3)
  M031/1(LL1) -> Eval30/1(In1)
  M031/2(LL2) -> Eval30/2(In2)
  M031/3(LL3) -> Eval30/3(In3)
  Eval30/1(Out1) -> To Workspace30/1
  [in1] -> M032/1(CT1)
  [in5] -> M032/2(T1)
  [in6] -> M032/3(EB1)
  [in7] -> M032/4(CT2)
  [in8] -> M032/5(F2)
  [in9] -> M032/6(E2)
  [in10] -> M032/7(MR2)
  [in11] -> M032/8(T2)
  [in12] -> M032/9(EB2)
  [in13] -> M032/10(CT3)
  [in17] -> M032/11(T3)
  [in18] -> M032/12(EB3)
  M032/1(LL1) -> Eval31/1(In1)
  M032/2(LL2) -> Eval31/2(In2)
  M032/3(LL3) -> Eval31/3(In3)
  Eval31/1(Out1) -> To Workspace31/1
  [in1] -> M033/1(CT1)
  [in5] -> M033/2(T1)
  [in6] -> M033/3(EB1)
  [in7] -> M033/4(CT2)
  [in8] -> M033/5(F2)
  [in9] -> M033/6(E2)
  [in10] -> M033/7(MR2)
  [in11] -> M033/8(T2)
  [in12] -> M033/9(EB2)
  [in13] -> M033/10(CT3)
  [in17] -> M033/11(T3)
  [in18] -> M033/12(EB3)
  M033/1(LL1) -> Eval32/1(In1)
  M033/2(LL2) -> Eval32/2(In2)
  M033/3(LL3) -> Eval32/3(In3)
  Eval32/1(Out1) -> To Workspace32/1
  [in1] -> M034/1(CT1)
  [in5] -> M034/2(T1)
  [in6] -> M034/3(EB1)
  [in7] -> M034/4(CT2)
  [in8] -> M034/5(F2)
  [in9] -> M034/6(E2)
  [in10] -> M034/7(MR2)
  [in11] -> M034/8(T2)
  [in12] -> M034/9(EB2)
  [in13] -> M034/10(CT3)
  [in17] -> M034/11(T3)
  [in18] -> M034/12(EB3)
  M034/1(LL1) -> Eval33/1(In1)
  M034/2(LL2) -> Eval33/2(In2)
  M034/3(LL3) -> Eval33/3(In3)
  Eval33/1(Out1) -> To Workspace33/1
  [in1] -> M035/1(CT1)
  [in5] -> M035/2(T1)
  [in6] -> M035/3(EB1)
  [in7] -> M035/4(CT2)
  [in8] -> M035/5(F2)
  [in9] -> M035/6(E2)
  [in10] -> M035/7(MR2)
  [in11] -> M035/8(T2)
  [in12] -> M035/9(EB2)
  [in13] -> M035/10(CT3)
  [in17] -> M035/11(T3)
  [in18] -> M035/12(EB3)
  M035/1(LL1) -> Eval34/1(In1)
  M035/2(LL2) -> Eval34/2(In2)
  M035/3(LL3) -> Eval34/3(In3)
  Eval34/1(Out1) -> To Workspace34/1
  [in1] -> M057/1(CT1)
  [in5] -> M057/2(T1)
  [in6] -> M057/3(EB1)
  [in7] -> M057/4(CT2)
  [in8] -> M057/5(F2)
  [in9] -> M057/6(E2)
  [in10] -> M057/7(MR2)
  [in11] -> M057/8(T2)
  [in12] -> M057/9(EB2)
  [in13] -> M057/10(CT3)
  [in17] -> M057/11(T3)
  [in18] -> M057/12(EB3)
  M057/1(LL1) -> Eval56/1(In1)
  M057/2(LL2) -> Eval56/2(In2)
  M057/3(LL3) -> Eval56/3(In3)
  Eval56/1(Out1) -> To Workspace56/1
  [in1] -> M058/1(CT1)
  [in5] -> M058/2(T1)
  [in6] -> M058/3(EB1)
  [in7] -> M058/4(CT2)
  [in8] -> M058/5(F2)
  [in9] -> M058/6(E2)
  [in10] -> M058/7(MR2)
  [in11] -> M058/8(T2)
  [in12] -> M058/9(EB2)
  [in13] -> M058/10(CT3)
  [in17] -> M058/11(T3)
  [in18] -> M058/12(EB3)
  M058/1(LL1) -> Eval57/1(In1)
  M058/2(LL2) -> Eval57/2(In2)
  M058/3(LL3) -> Eval57/3(In3)
  Eval57/1(Out1) -> To Workspace57/1
  [in1] -> M059/1(CT1)
  [in5] -> M059/2(T1)
  [in6] -> M059/3(EB1)
  [in7] -> M059/4(CT2)
  [in8] -> M059/5(F2)
  [in9] -> M059/6(E2)
  [in10] -> M059/7(MR2)
  [in11] -> M059/8(T2)
  [in12] -> M059/9(EB2)
  [in13] -> M059/10(CT3)
  [in17] -> M059/11(T3)
  [in18] -> M059/12(EB3)
  M059/1(LL1) -> Eval58/1(In1)
  M059/2(LL2) -> Eval58/2(In2)
  M059/3(LL3) -> Eval58/3(In3)
  Eval58/1(Out1) -> To Workspace58/1
  [in1] -> M060/1(CT1)
  [in5] -> M060/2(T1)
  [in6] -> M060/3(EB1)
  [in7] -> M060/4(CT2)
  [in8] -> M060/5(F2)
  [in9] -> M060/6(E2)
  [in10] -> M060/7(MR2)
  [in11] -> M060/8(T2)
  [in12] -> M060/9(EB2)
  [in13] -> M060/10(CT3)
  [in17] -> M060/11(T3)
  [in18] -> M060/12(EB3)
  M060/1(LL1) -> Eval59/1(In1)
  M060/2(LL2) -> Eval59/2(In2)
  M060/3(LL3) -> Eval59/3(In3)
  Eval59/1(Out1) -> To Workspace59/1
  [in1] -> M061/1(CT1)
  [in5] -> M061/2(T1)
  [in6] -> M061/3(EB1)
  [in7] -> M061/4(CT2)
  [in8] -> M061/5(F2)
  [in9] -> M061/6(E2)
  [in10] -> M061/7(MR2)
  [in11] -> M061/8(T2)
  [in12] -> M061/9(EB2)
  [in13] -> M061/10(CT3)
  [in17] -> M061/11(T3)
  [in18] -> M061/12(EB3)
  M061/1(LL1) -> Eval60/1(In1)
  M061/2(LL2) -> Eval60/2(In2)
  M061/3(LL3) -> Eval60/3(In3)
  Eval60/1(Out1) -> To Workspace60/1
  [in1] -> M062/1(CT1)
  [in5] -> M062/2(T1)
  [in6] -> M062/3(EB1)
  [in7] -> M062/4(CT2)
  [in8] -> M062/5(F2)
  [in9] -> M062/6(E2)
  [in10] -> M062/7(MR2)
  [in11] -> M062/8(T2)
  [in12] -> M062/9(EB2)
  [in13] -> M062/10(CT3)
  [in17] -> M062/11(T3)
  [in18] -> M062/12(EB3)
  M062/1(LL1) -> Eval61/1(In1)
  M062/2(LL2) -> Eval61/2(In2)
  M062/3(LL3) -> Eval61/3(In3)
  Eval61/1(Out1) -> To Workspace61/1
  [in1] -> M063/1(CT1)
  [in5] -> M063/2(T1)
  [in6] -> M063/3(EB1)
  [in7] -> M063/4(CT2)
  [in8] -> M063/5(F2)
  [in9] -> M063/6(E2)
  [in10] -> M063/7(MR2)
  [in11] -> M063/8(T2)
  [in12] -> M063/9(EB2)
  [in13] -> M063/10(CT3)
  [in17] -> M063/11(T3)
  [in18] -> M063/12(EB3)
  M063/1(LL1) -> Eval62/1(In1)
  M063/2(LL2) -> Eval62/2(In2)
  M063/3(LL3) -> Eval62/3(In3)
  Eval62/1(Out1) -> To Workspace62/1
  [in1] -> M064/1(CT1)
  [in5] -> M064/2(T1)
  [in6] -> M064/3(EB1)
  [in7] -> M064/4(CT2)
  [in8] -> M064/5(F2)
  [in9] -> M064/6(E2)
  [in10] -> M064/7(MR2)
  [in11] -> M064/8(T2)
  [in12] -> M064/9(EB2)
  [in13] -> M064/10(CT3)
  [in17] -> M064/11(T3)
  [in18] -> M064/12(EB3)
  M064/1(LL1) -> Eval63/1(In1)
  M064/2(LL2) -> Eval63/2(In2)
  M064/3(LL3) -> Eval63/3(In3)
  Eval63/1(Out1) -> To Workspace63/1
  [in1] -> M065/1(CT1)
  [in5] -> M065/2(T1)
  [in6] -> M065/3(EB1)
  [in7] -> M065/4(CT2)
  [in8] -> M065/5(F2)
  [in9] -> M065/6(E2)
  [in10] -> M065/7(MR2)
  [in11] -> M065/8(T2)
  [in12] -> M065/9(EB2)
  [in13] -> M065/10(CT3)
  [in17] -> M065/11(T3)
  [in18] -> M065/12(EB3)
  M065/1(LL1) -> Eval64/1(In1)
  M065/2(LL2) -> Eval64/2(In2)
  M065/3(LL3) -> Eval64/3(In3)
  Eval64/1(Out1) -> To Workspace64/1
  [in1] -> M066/1(CT1)
  [in5] -> M066/2(T1)
  [in6] -> M066/3(EB1)
  [in7] -> M066/4(CT2)
  [in8] -> M066/5(F2)
  [in9] -> M066/6(E2)
  [in10] -> M066/7(MR2)
  [in11] -> M066/8(T2)
  [in12] -> M066/9(EB2)
  [in13] -> M066/10(CT3)
  [in17] -> M066/11(T3)
  [in18] -> M066/12(EB3)
  M066/1(LL1) -> Eval65/1(In1)
  M066/2(LL2) -> Eval65/2(In2)
  M066/3(LL3) -> Eval65/3(In3)
  Eval65/1(Out1) -> To Workspace65/1
  [in1] -> M067/1(CT1)
  [in5] -> M067/2(T1)
  [in6] -> M067/3(EB1)
  [in7] -> M067/4(CT2)
  [in8] -> M067/5(F2)
  [in9] -> M067/6(E2)
  [in10] -> M067/7(MR2)
  [in11] -> M067/8(T2)
  [in12] -> M067/9(EB2)
  [in13] -> M067/10(CT3)
  [in17] -> M067/11(T3)
  [in18] -> M067/12(EB3)
  M067/1(LL1) -> Eval66/1(In1)
  M067/2(LL2) -> Eval66/2(In2)
  M067/3(LL3) -> Eval66/3(In3)
  Eval66/1(Out1) -> To Workspace66/1
  [in1] -> M068/1(CT1)
  [in5] -> M068/2(T1)
  [in6] -> M068/3(EB1)
  [in7] -> M068/4(CT2)
  [in8] -> M068/5(F2)
  [in9] -> M068/6(E2)
  [in10] -> M068/7(MR2)
  [in11] -> M068/8(T2)
  [in12] -> M068/9(EB2)
  [in13] -> M068/10(CT3)
  [in17] -> M068/11(T3)
  [in18] -> M068/12(EB3)
  M068/1(LL1) -> Eval67/1(In1)
  M068/2(LL2) -> Eval67/2(In2)
  M068/3(LL3) -> Eval67/3(In3)
  Eval67/1(Out1) -> To Workspace67/1
  [in1] -> M069/1(CT1)
  [in5] -> M069/2(T1)
  [in6] -> M069/3(EB1)
  [in7] -> M069/4(CT2)
  [in8] -> M069/5(F2)
  [in9] -> M069/6(E2)
  [in10] -> M069/7(MR2)
  [in11] -> M069/8(T2)
  [in12] -> M069/9(EB2)
  [in13] -> M069/10(CT3)
  [in17] -> M069/11(T3)
  [in18] -> M069/12(EB3)
  M069/1(LL1) -> Eval68/1(In1)
  M069/2(LL2) -> Eval68/2(In2)
  M069/3(LL3) -> Eval68/3(In3)
  Eval68/1(Out1) -> To Workspace68/1
  [in1] -> M070/1(CT1)
  [in5] -> M070/2(T1)
  [in6] -> M070/3(EB1)
  [in7] -> M070/4(CT2)
  [in8] -> M070/5(F2)
  [in9] -> M070/6(E2)
  [in10] -> M070/7(MR2)
  [in11] -> M070/8(T2)
  [in12] -> M070/9(EB2)
  [in13] -> M070/10(CT3)
  [in17] -> M070/11(T3)
  [in18] -> M070/12(EB3)
  M070/1(LL1) -> Eval69/1(In1)
  M070/2(LL2) -> Eval69/2(In2)
  M070/3(LL3) -> Eval69/3(In3)
  Eval69/1(Out1) -> To Workspace69/1
  [in1] -> M071/1(CT1)
  [in5] -> M071/2(T1)
  [in6] -> M071/3(EB1)
  [in7] -> M071/4(CT2)
  [in8] -> M071/5(F2)
  [in9] -> M071/6(E2)
  [in10] -> M071/7(MR2)
  [in11] -> M071/8(T2)
  [in12] -> M071/9(EB2)
  [in13] -> M071/10(CT3)
  [in17] -> M071/11(T3)
  [in18] -> M071/12(EB3)
  M071/1(LL1) -> Eval70/1(In1)
  M071/2(LL2) -> Eval70/2(In2)
  M071/3(LL3) -> Eval70/3(In3)
  Eval70/1(Out1) -> To Workspace70/1
  [in1] -> M072/1(CT1)
  [in5] -> M072/2(T1)
  [in6] -> M072/3(EB1)
  [in7] -> M072/4(CT2)
  [in8] -> M072/5(F2)
  [in9] -> M072/6(E2)
  [in10] -> M072/7(MR2)
  [in11] -> M072/8(T2)
  [in12] -> M072/9(EB2)
  [in13] -> M072/10(CT3)
  [in17] -> M072/11(T3)
  [in18] -> M072/12(EB3)
  M072/1(LL1) -> Eval71/1(In1)
  M072/2(LL2) -> Eval71/2(In2)
  M072/3(LL3) -> Eval71/3(In3)
  Eval71/1(Out1) -> To Workspace71/1
  [in1] -> M073/1(CT1)
  [in5] -> M073/2(T1)
  [in6] -> M073/3(EB1)
  [in7] -> M073/4(CT2)
  [in8] -> M073/5(F2)
  [in9] -> M073/6(E2)
  [in10] -> M073/7(MR2)
  [in11] -> M073/8(T2)
  [in12] -> M073/9(EB2)
  [in13] -> M073/10(CT3)
  [in17] -> M073/11(T3)
  [in18] -> M073/12(EB3)
  M073/1(LL1) -> Eval72/1(In1)
  M073/2(LL2) -> Eval72/2(In2)
  M073/3(LL3) -> Eval72/3(In3)
  Eval72/1(Out1) -> To Workspace72/1
  [in1] -> M074/1(CT1)
  [in5] -> M074/2(T1)
  [in6] -> M074/3(EB1)
  [in7] -> M074/4(CT2)
  [in8] -> M074/5(F2)
  [in9] -> M074/6(E2)
  [in10] -> M074/7(MR2)
  [in11] -> M074/8(T2)
  [in12] -> M074/9(EB2)
  [in13] -> M074/10(CT3)
  [in17] -> M074/11(T3)
  [in18] -> M074/12(EB3)
  M074/1(LL1) -> Eval73/1(In1)
  M074/2(LL2) -> Eval73/2(In2)
  M074/3(LL3) -> Eval73/3(In3)
  Eval73/1(Out1) -> To Workspace73/1
  [in1] -> M075/1(CT1)
  [in5] -> M075/2(T1)
  [in6] -> M075/3(EB1)
  [in7] -> M075/4(CT2)
  [in8] -> M075/5(F2)
  [in9] -> M075/6(E2)
  [in10] -> M075/7(MR2)
  [in11] -> M075/8(T2)
  [in12] -> M075/9(EB2)
  [in13] -> M075/10(CT3)
  [in17] -> M075/11(T3)
  [in18] -> M075/12(EB3)
  M075/1(LL1) -> Eval74/1(In1)
  M075/2(LL2) -> Eval74/2(In2)
  M075/3(LL3) -> Eval74/3(In3)
  Eval74/1(Out1) -> To Workspace74/1
  [in1] -> M076/1(CT1)
  [in5] -> M076/2(T1)
  [in6] -> M076/3(EB1)
  [in7] -> M076/4(CT2)
  [in8] -> M076/5(F2)
  [in9] -> M076/6(E2)
  [in10] -> M076/7(MR2)
  [in11] -> M076/8(T2)
  [in12] -> M076/9(EB2)
  [in13] -> M076/10(CT3)
  [in17] -> M076/11(T3)
  [in18] -> M076/12(EB3)
  M076/1(LL1) -> Eval75/1(In1)
  M076/2(LL2) -> Eval75/2(In2)
  M076/3(LL3) -> Eval75/3(In3)
  Eval75/1(Out1) -> To Workspace75/1
  [in1] -> M077/1(CT1)
  [in5] -> M077/2(T1)
  [in6] -> M077/3(EB1)
  [in7] -> M077/4(CT2)
  [in8] -> M077/5(F2)
  [in9] -> M077/6(E2)
  [in10] -> M077/7(MR2)
  [in11] -> M077/8(T2)
  [in12] -> M077/9(EB2)
  [in13] -> M077/10(CT3)
  [in17] -> M077/11(T3)
  [in18] -> M077/12(EB3)
  M077/1(LL1) -> Eval76/1(In1)
  M077/2(LL2) -> Eval76/2(In2)
  M077/3(LL3) -> Eval76/3(In3)
  Eval76/1(Out1) -> To Workspace76/1
  [in1] -> M078/1(CT1)
  [in5] -> M078/2(T1)
  [in6] -> M078/3(EB1)
  [in7] -> M078/4(CT2)
  [in8] -> M078/5(F2)
  [in9] -> M078/6(E2)
  [in10] -> M078/7(MR2)
  [in11] -> M078/8(T2)
  [in12] -> M078/9(EB2)
  [in13] -> M078/10(CT3)
  [in17] -> M078/11(T3)
  [in18] -> M078/12(EB3)
  M078/1(LL1) -> Eval77/1(In1)
  M078/2(LL2) -> Eval77/2(In2)
  M078/3(LL3) -> Eval77/3(In3)
  Eval77/1(Out1) -> To Workspace77/1
  [in1] -> M079/1(CT1)
  [in5] -> M079/2(T1)
  [in6] -> M079/3(EB1)
  [in7] -> M079/4(CT2)
  [in8] -> M079/5(F2)
  [in9] -> M079/6(E2)
  [in10] -> M079/7(MR2)
  [in11] -> M079/8(T2)
  [in12] -> M079/9(EB2)
  [in13] -> M079/10(CT3)
  [in17] -> M079/11(T3)
  [in18] -> M079/12(EB3)
  M079/1(LL1) -> Eval78/1(In1)
  M079/2(LL2) -> Eval78/2(In2)
  M079/3(LL3) -> Eval78/3(In3)
  Eval78/1(Out1) -> To Workspace78/1
  [in1] -> M080/1(CT1)
  [in5] -> M080/2(T1)
  [in6] -> M080/3(EB1)
  [in7] -> M080/4(CT2)
  [in8] -> M080/5(F2)
  [in9] -> M080/6(E2)
  [in10] -> M080/7(MR2)
  [in11] -> M080/8(T2)
  [in12] -> M080/9(EB2)
  [in13] -> M080/10(CT3)
  [in17] -> M080/11(T3)
  [in18] -> M080/12(EB3)
  M080/1(LL1) -> Eval79/1(In1)
  M080/2(LL2) -> Eval79/2(In2)
  M080/3(LL3) -> Eval79/3(In3)
  Eval79/1(Out1) -> To Workspace79/1
  [in1] -> M081/1(CT1)
  [in5] -> M081/2(T1)
  [in6] -> M081/3(EB1)
  [in7] -> M081/4(CT2)
  [in8] -> M081/5(F2)
  [in9] -> M081/6(E2)
  [in10] -> M081/7(MR2)
  [in11] -> M081/8(T2)
  [in12] -> M081/9(EB2)
  [in13] -> M081/10(CT3)
  [in17] -> M081/11(T3)
  [in18] -> M081/12(EB3)
  M081/1(LL1) -> Eval80/1(In1)
  M081/2(LL2) -> Eval80/2(In2)
  M081/3(LL3) -> Eval80/3(In3)
  Eval80/1(Out1) -> To Workspace80/1
  [in1] -> M082/1(CT1)
  [in5] -> M082/2(T1)
  [in6] -> M082/3(EB1)
  [in7] -> M082/4(CT2)
  [in8] -> M082/5(F2)
  [in9] -> M082/6(E2)
  [in10] -> M082/7(MR2)
  [in11] -> M082/8(T2)
  [in12] -> M082/9(EB2)
  [in13] -> M082/10(CT3)
  [in17] -> M082/11(T3)
  [in18] -> M082/12(EB3)
  M082/1(LL1) -> Eval81/1(In1)
  M082/2(LL2) -> Eval81/2(In2)
  M082/3(LL3) -> Eval81/3(In3)
  Eval81/1(Out1) -> To Workspace81/1
  [in1] -> M083/1(CT1)
  [in5] -> M083/2(T1)
  [in6] -> M083/3(EB1)
  [in7] -> M083/4(CT2)
  [in8] -> M083/5(F2)
  [in9] -> M083/6(E2)
  [in10] -> M083/7(MR2)
  [in11] -> M083/8(T2)
  [in12] -> M083/9(EB2)
  [in13] -> M083/10(CT3)
  [in17] -> M083/11(T3)
  [in18] -> M083/12(EB3)
  M083/1(LL1) -> Eval82/1(In1)
  M083/2(LL2) -> Eval82/2(In2)
  M083/3(LL3) -> Eval82/3(In3)
  Eval82/1(Out1) -> To Workspace82/1
  [in1] -> M084/1(CT1)
  [in5] -> M084/2(T1)
  [in6] -> M084/3(EB1)
  [in7] -> M084/4(CT2)
  [in8] -> M084/5(F2)
  [in9] -> M084/6(E2)
  [in10] -> M084/7(MR2)
  [in11] -> M084/8(T2)
  [in12] -> M084/9(EB2)
  [in13] -> M084/10(CT3)
  [in17] -> M084/11(T3)
  [in18] -> M084/12(EB3)
  M084/1(LL1) -> Eval83/1(In1)
  M084/2(LL2) -> Eval83/2(In2)
  M084/3(LL3) -> Eval83/3(In3)
  Eval83/1(Out1) -> To Workspace83/1
  [in1] -> M085/1(CT1)
  [in5] -> M085/2(T1)
  [in6] -> M085/3(EB1)
  [in7] -> M085/4(CT2)
  [in8] -> M085/5(F2)
  [in9] -> M085/6(E2)
  [in10] -> M085/7(MR2)
  [in11] -> M085/8(T2)
  [in12] -> M085/9(EB2)
  [in13] -> M085/10(CT3)
  [in17] -> M085/11(T3)
  [in18] -> M085/12(EB3)
  M085/1(LL1) -> Eval84/1(In1)
  M085/2(LL2) -> Eval84/2(In2)
  M085/3(LL3) -> Eval84/3(In3)
  Eval84/1(Out1) -> To Workspace84/1
  [in1] -> M086/1(CT1)
  [in5] -> M086/2(T1)
  [in6] -> M086/3(EB1)
  [in7] -> M086/4(CT2)
  [in8] -> M086/5(F2)
  [in9] -> M086/6(E2)
  [in10] -> M086/7(MR2)
  [in11] -> M086/8(T2)
  [in12] -> M086/9(EB2)
  [in13] -> M086/10(CT3)
  [in17] -> M086/11(T3)
  [in18] -> M086/12(EB3)
  M086/1(LL1) -> Eval85/1(In1)
  M086/2(LL2) -> Eval85/2(In2)
  M086/3(LL3) -> Eval85/3(In3)
  Eval85/1(Out1) -> To Workspace85/1
  [in1] -> M087/1(CT1)
  [in5] -> M087/2(T1)
  [in6] -> M087/3(EB1)
  [in7] -> M087/4(CT2)
  [in8] -> M087/5(F2)
  [in9] -> M087/6(E2)
  [in10] -> M087/7(MR2)
  [in11] -> M087/8(T2)
  [in12] -> M087/9(EB2)
  [in13] -> M087/10(CT3)
  [in17] -> M087/11(T3)
  [in18] -> M087/12(EB3)
  M087/1(LL1) -> Eval86/1(In1)
  M087/2(LL2) -> Eval86/2(In2)
  M087/3(LL3) -> Eval86/3(In3)
  Eval86/1(Out1) -> To Workspace86/1
  [in1] -> M088/1(CT1)
  [in5] -> M088/2(T1)
  [in6] -> M088/3(EB1)
  [in7] -> M088/4(CT2)
  [in8] -> M088/5(F2)
  [in9] -> M088/6(E2)
  [in10] -> M088/7(MR2)
  [in11] -> M088/8(T2)
  [in12] -> M088/9(EB2)
  [in13] -> M088/10(CT3)
  [in17] -> M088/11(T3)
  [in18] -> M088/12(EB3)
  M088/1(LL1) -> Eval87/1(In1)
  M088/2(LL2) -> Eval87/2(In2)
  M088/3(LL3) -> Eval87/3(In3)
  Eval87/1(Out1) -> To Workspace87/1
  [in1] -> M089/1(CT1)
  [in5] -> M089/2(T1)
  [in6] -> M089/3(EB1)
  [in7] -> M089/4(CT2)
  [in8] -> M089/5(F2)
  [in9] -> M089/6(E2)
  [in10] -> M089/7(MR2)
  [in11] -> M089/8(T2)
  [in12] -> M089/9(EB2)
  [in13] -> M089/10(CT3)
  [in17] -> M089/11(T3)
  [in18] -> M089/12(EB3)
  M089/1(LL1) -> Eval88/1(In1)
  M089/2(LL2) -> Eval88/2(In2)
  M089/3(LL3) -> Eval88/3(In3)
  Eval88/1(Out1) -> To Workspace88/1
  [in1] -> M090/1(CT1)
  [in5] -> M090/2(T1)
  [in6] -> M090/3(EB1)
  [in7] -> M090/4(CT2)
  [in8] -> M090/5(F2)
  [in9] -> M090/6(E2)
  [in10] -> M090/7(MR2)
  [in11] -> M090/8(T2)
  [in12] -> M090/9(EB2)
  [in13] -> M090/10(CT3)
  [in17] -> M090/11(T3)
  [in18] -> M090/12(EB3)
  M090/1(LL1) -> Eval89/1(In1)
  M090/2(LL2) -> Eval89/2(In2)
  M090/3(LL3) -> Eval89/3(In3)
  Eval89/1(Out1) -> To Workspace89/1
  [in1] -> M091/1(CT1)
  [in5] -> M091/2(T1)
  [in6] -> M091/3(EB1)
  [in7] -> M091/4(CT2)
  [in8] -> M091/5(F2)
  [in9] -> M091/6(E2)
  [in10] -> M091/7(MR2)
  [in11] -> M091/8(T2)
  [in12] -> M091/9(EB2)
  [in13] -> M091/10(CT3)
  [in17] -> M091/11(T3)
  [in18] -> M091/12(EB3)
  M091/1(LL1) -> Eval90/1(In1)
  M091/2(LL2) -> Eval90/2(In2)
  M091/3(LL3) -> Eval90/3(In3)
  Eval90/1(Out1) -> To Workspace90/1
  [in1] -> M092/1(CT1)
  [in5] -> M092/2(T1)
  [in6] -> M092/3(EB1)
  [in7] -> M092/4(CT2)
  [in8] -> M092/5(F2)
  [in9] -> M092/6(E2)
  [in10] -> M092/7(MR2)
  [in11] -> M092/8(T2)
  [in12] -> M092/9(EB2)
  [in13] -> M092/10(CT3)
  [in17] -> M092/11(T3)
  [in18] -> M092/12(EB3)
  M092/1(LL1) -> Eval91/1(In1)
  M092/2(LL2) -> Eval91/2(In2)
  M092/3(LL3) -> Eval91/3(In3)
  Eval91/1(Out1) -> To Workspace91/1
  [in1] -> M093/1(CT1)
  [in5] -> M093/2(T1)
  [in6] -> M093/3(EB1)
  [in7] -> M093/4(CT2)
  [in8] -> M093/5(F2)
  [in9] -> M093/6(E2)
  [in10] -> M093/7(MR2)
  [in11] -> M093/8(T2)
  [in12] -> M093/9(EB2)
  [in13] -> M093/10(CT3)
  [in17] -> M093/11(T3)
  [in18] -> M093/12(EB3)
  M093/1(LL1) -> Eval92/1(In1)
  M093/2(LL2) -> Eval92/2(In2)
  M093/3(LL3) -> Eval92/3(In3)
  Eval92/1(Out1) -> To Workspace92/1
  [in1] -> M094/1(CT1)
  [in5] -> M094/2(T1)
  [in6] -> M094/3(EB1)
  [in7] -> M094/4(CT2)
  [in8] -> M094/5(F2)
  [in9] -> M094/6(E2)
  [in10] -> M094/7(MR2)
  [in11] -> M094/8(T2)
  [in12] -> M094/9(EB2)
  [in13] -> M094/10(CT3)
  [in17] -> M094/11(T3)
  [in18] -> M094/12(EB3)
  M094/1(LL1) -> Eval93/1(In1)
  M094/2(LL2) -> Eval93/2(In2)
  M094/3(LL3) -> Eval93/3(In3)
  Eval93/1(Out1) -> To Workspace93/1
  [in1] -> M095/1(CT1)
  [in5] -> M095/2(T1)
  [in6] -> M095/3(EB1)
  [in7] -> M095/4(CT2)
  [in8] -> M095/5(F2)
  [in9] -> M095/6(E2)
  [in10] -> M095/7(MR2)
  [in11] -> M095/8(T2)
  [in12] -> M095/9(EB2)
  [in13] -> M095/10(CT3)
  [in17] -> M095/11(T3)
  [in18] -> M095/12(EB3)
  M095/1(LL1) -> Eval94/1(In1)
  M095/2(LL2) -> Eval94/2(In2)
  M095/3(LL3) -> Eval94/3(In3)
  Eval94/1(Out1) -> To Workspace94/1
  [in1] -> M096/1(CT1)
  [in5] -> M096/2(T1)
  [in6] -> M096/3(EB1)
  [in7] -> M096/4(CT2)
  [in8] -> M096/5(F2)
  [in9] -> M096/6(E2)
  [in10] -> M096/7(MR2)
  [in11] -> M096/8(T2)
  [in12] -> M096/9(EB2)
  [in13] -> M096/10(CT3)
  [in17] -> M096/11(T3)
  [in18] -> M096/12(EB3)
  M096/1(LL1) -> Eval95/1(In1)
  M096/2(LL2) -> Eval95/2(In2)
  M096/3(LL3) -> Eval95/3(In3)
  Eval95/1(Out1) -> To Workspace95/1
  [in1] -> M097/1(CT1)
  [in5] -> M097/2(T1)
  [in6] -> M097/3(EB1)
  [in7] -> M097/4(CT2)
  [in8] -> M097/5(F2)
  [in9] -> M097/6(E2)
  [in10] -> M097/7(MR2)
  [in11] -> M097/8(T2)
  [in12] -> M097/9(EB2)
  [in13] -> M097/10(CT3)
  [in17] -> M097/11(T3)
  [in18] -> M097/12(EB3)
  M097/1(LL1) -> Eval96/1(In1)
  M097/2(LL2) -> Eval96/2(In2)
  M097/3(LL3) -> Eval96/3(In3)
  Eval96/1(Out1) -> To Workspace96/1
  [in1] -> M098/1(CT1)
  [in5] -> M098/2(T1)
  [in6] -> M098/3(EB1)
  [in7] -> M098/4(CT2)
  [in8] -> M098/5(F2)
  [in9] -> M098/6(E2)
  [in10] -> M098/7(MR2)
  [in11] -> M098/8(T2)
  [in12] -> M098/9(EB2)
  [in13] -> M098/10(CT3)
  [in17] -> M098/11(T3)
  [in18] -> M098/12(EB3)
  M098/1(LL1) -> Eval97/1(In1)
  M098/2(LL2) -> Eval97/2(In2)
  M098/3(LL3) -> Eval97/3(In3)
  Eval97/1(Out1) -> To Workspace97/1
  [in1] -> M099/1(CT1)
  [in5] -> M099/2(T1)
  [in6] -> M099/3(EB1)
  [in7] -> M099/4(CT2)
  [in8] -> M099/5(F2)
  [in9] -> M099/6(E2)
  [in10] -> M099/7(MR2)
  [in11] -> M099/8(T2)
  [in12] -> M099/9(EB2)
  [in13] -> M099/10(CT3)
  [in17] -> M099/11(T3)
  [in18] -> M099/12(EB3)
  M099/1(LL1) -> Eval98/1(In1)
  M099/2(LL2) -> Eval98/2(In2)
  M099/3(LL3) -> Eval98/3(In3)
  Eval98/1(Out1) -> To Workspace98/1
  [in1] -> M100/1(CT1)
  [in5] -> M100/2(T1)
  [in6] -> M100/3(EB1)
  [in7] -> M100/4(CT2)
  [in8] -> M100/5(F2)
  [in9] -> M100/6(E2)
  [in10] -> M100/7(MR2)
  [in11] -> M100/8(T2)
  [in12] -> M100/9(EB2)
  [in13] -> M100/10(CT3)
  [in17] -> M100/11(T3)
  [in18] -> M100/12(EB3)
  M100/1(LL1) -> Eval99/1(In1)
  M100/2(LL2) -> Eval99/2(In2)
  M100/3(LL3) -> Eval99/3(In3)
  Eval99/1(Out1) -> To Workspace99/1
  [in1] -> M101/1(CT1)
  [in5] -> M101/2(T1)
  [in6] -> M101/3(EB1)
  [in7] -> M101/4(CT2)
  [in8] -> M101/5(F2)
  [in9] -> M101/6(E2)
  [in10] -> M101/7(MR2)
  [in11] -> M101/8(T2)
  [in12] -> M101/9(EB2)
  [in13] -> M101/10(CT3)
  [in17] -> M101/11(T3)
  [in18] -> M101/12(EB3)
  M101/1(LL1) -> Eval100/1(In1)
  M101/2(LL2) -> Eval100/2(In2)
  M101/3(LL3) -> Eval100/3(In3)
  Eval100/1(Out1) -> To Workspace100/1
  [in1] -> M102/1(CT1)
  [in5] -> M102/2(T1)
  [in6] -> M102/3(EB1)
  [in7] -> M102/4(CT2)
  [in8] -> M102/5(F2)
  [in9] -> M102/6(E2)
  [in10] -> M102/7(MR2)
  [in11] -> M102/8(T2)
  [in12] -> M102/9(EB2)
  [in13] -> M102/10(CT3)
  [in17] -> M102/11(T3)
  [in18] -> M102/12(EB3)
  M102/1(LL1) -> Eval101/1(In1)
  M102/2(LL2) -> Eval101/2(In2)
  M102/3(LL3) -> Eval101/3(In3)
  Eval101/1(Out1) -> To Workspace101/1
  [in1] -> M103/1(CT1)
  [in5] -> M103/2(T1)
  [in6] -> M103/3(EB1)
  [in7] -> M103/4(CT2)
  [in8] -> M103/5(F2)
  [in9] -> M103/6(E2)
  [in10] -> M103/7(MR2)
  [in11] -> M103/8(T2)
  [in12] -> M103/9(EB2)
  [in13] -> M103/10(CT3)
  [in17] -> M103/11(T3)
  [in18] -> M103/12(EB3)
  M103/1(LL1) -> Eval102/1(In1)
  M103/2(LL2) -> Eval102/2(In2)
  M103/3(LL3) -> Eval102/3(In3)
  Eval102/1(Out1) -> To Workspace102/1
  [in1] -> M104/1(CT1)
  [in5] -> M104/2(T1)
  [in6] -> M104/3(EB1)
  [in7] -> M104/4(CT2)
  [in8] -> M104/5(F2)
  [in9] -> M104/6(E2)
  [in10] -> M104/7(MR2)
  [in11] -> M104/8(T2)
  [in12] -> M104/9(EB2)
  [in13] -> M104/10(CT3)
  [in17] -> M104/11(T3)
  [in18] -> M104/12(EB3)
  M104/1(LL1) -> Eval103/1(In1)
  M104/2(LL2) -> Eval103/2(In2)
  M104/3(LL3) -> Eval103/3(In3)
  Eval103/1(Out1) -> To Workspace103/1
  [in1] -> M105/1(CT1)
  [in5] -> M105/2(T1)
  [in6] -> M105/3(EB1)
  [in7] -> M105/4(CT2)
  [in8] -> M105/5(F2)
  [in9] -> M105/6(E2)
  [in10] -> M105/7(MR2)
  [in11] -> M105/8(T2)
  [in12] -> M105/9(EB2)
  [in13] -> M105/10(CT3)
  [in17] -> M105/11(T3)
  [in18] -> M105/12(EB3)
  M105/1(LL1) -> Eval104/1(In1)
  M105/2(LL2) -> Eval104/2(In2)
  M105/3(LL3) -> Eval104/3(In3)
  Eval104/1(Out1) -> To Workspace104/1
  [in1] -> M106/1(CT1)
  [in5] -> M106/2(T1)
  [in6] -> M106/3(EB1)
  [in7] -> M106/4(CT2)
  [in8] -> M106/5(F2)
  [in9] -> M106/6(E2)
  [in10] -> M106/7(MR2)
  [in11] -> M106/8(T2)
  [in12] -> M106/9(EB2)
  [in13] -> M106/10(CT3)
  [in17] -> M106/11(T3)
  [in18] -> M106/12(EB3)
  M106/1(LL1) -> Eval105/1(In1)
  M106/2(LL2) -> Eval105/2(In2)
  M106/3(LL3) -> Eval105/3(In3)
  Eval105/1(Out1) -> To Workspace105/1
  [in1] -> M107/1(CT1)
  [in5] -> M107/2(T1)
  [in6] -> M107/3(EB1)
  [in7] -> M107/4(CT2)
  [in8] -> M107/5(F2)
  [in9] -> M107/6(E2)
  [in10] -> M107/7(MR2)
  [in11] -> M107/8(T2)
  [in12] -> M107/9(EB2)
  [in13] -> M107/10(CT3)
  [in17] -> M107/11(T3)
  [in18] -> M107/12(EB3)
  M107/1(LL1) -> Eval106/1(In1)
  M107/2(LL2) -> Eval106/2(In2)
  M107/3(LL3) -> Eval106/3(In3)
  Eval106/1(Out1) -> To Workspace106/1
  [in1] -> M108/1(CT1)
  [in5] -> M108/2(T1)
  [in6] -> M108/3(EB1)
  [in7] -> M108/4(CT2)
  [in8] -> M108/5(F2)
  [in9] -> M108/6(E2)
  [in10] -> M108/7(MR2)
  [in11] -> M108/8(T2)
  [in12] -> M108/9(EB2)
  [in13] -> M108/10(CT3)
  [in17] -> M108/11(T3)
  [in18] -> M108/12(EB3)
  M108/1(LL1) -> Eval107/1(In1)
  M108/2(LL2) -> Eval107/2(In2)
  M108/3(LL3) -> Eval107/3(In3)
  Eval107/1(Out1) -> To Workspace107/1
  [in1] -> M109/1(CT1)
  [in5] -> M109/2(T1)
  [in6] -> M109/3(EB1)
  [in7] -> M109/4(CT2)
  [in8] -> M109/5(F2)
  [in9] -> M109/6(E2)
  [in10] -> M109/7(MR2)
  [in11] -> M109/8(T2)
  [in12] -> M109/9(EB2)
  [in13] -> M109/10(CT3)
  [in17] -> M109/11(T3)
  [in18] -> M109/12(EB3)
  M109/1(LL1) -> Eval108/1(In1)
  M109/2(LL2) -> Eval108/2(In2)
  M109/3(LL3) -> Eval108/3(In3)
  Eval108/1(Out1) -> To Workspace108/1
  [in1] -> M110/1(CT1)
  [in5] -> M110/2(T1)
  [in6] -> M110/3(EB1)
  [in7] -> M110/4(CT2)
  [in8] -> M110/5(F2)
  [in9] -> M110/6(E2)
  [in10] -> M110/7(MR2)
  [in11] -> M110/8(T2)
  [in12] -> M110/9(EB2)
  [in13] -> M110/10(CT3)
  [in17] -> M110/11(T3)
  [in18] -> M110/12(EB3)
  M110/1(LL1) -> Eval109/1(In1)
  M110/2(LL2) -> Eval109/2(In2)
  M110/3(LL3) -> Eval109/3(In3)
  Eval109/1(Out1) -> To Workspace109/1
  [in1] -> M111/1(CT1)
  [in5] -> M111/2(T1)
  [in6] -> M111/3(EB1)
  [in7] -> M111/4(CT2)
  [in8] -> M111/5(F2)
  [in9] -> M111/6(E2)
  [in10] -> M111/7(MR2)
  [in11] -> M111/8(T2)
  [in12] -> M111/9(EB2)
  [in13] -> M111/10(CT3)
  [in17] -> M111/11(T3)
  [in18] -> M111/12(EB3)
  M111/1(LL1) -> Eval110/1(In1)
  M111/2(LL2) -> Eval110/2(In2)
  M111/3(LL3) -> Eval110/3(In3)
  Eval110/1(Out1) -> To Workspace110/1
  [in1] -> M112/1(CT1)
  [in5] -> M112/2(T1)
  [in6] -> M112/3(EB1)
  [in7] -> M112/4(CT2)
  [in8] -> M112/5(F2)
  [in9] -> M112/6(E2)
  [in10] -> M112/7(MR2)
  [in11] -> M112/8(T2)
  [in12] -> M112/9(EB2)
  [in13] -> M112/10(CT3)
  [in17] -> M112/11(T3)
  [in18] -> M112/12(EB3)
  M112/1(LL1) -> Eval111/1(In1)
  M112/2(LL2) -> Eval111/2(In2)
  M112/3(LL3) -> Eval111/3(In3)
  Eval111/1(Out1) -> To Workspace111/1
  [in1] -> M113/1(CT1)
  [in5] -> M113/2(T1)
  [in6] -> M113/3(EB1)
  [in7] -> M113/4(CT2)
  [in8] -> M113/5(F2)
  [in9] -> M113/6(E2)
  [in10] -> M113/7(MR2)
  [in11] -> M113/8(T2)
  [in12] -> M113/9(EB2)
  [in13] -> M113/10(CT3)
  [in17] -> M113/11(T3)
  [in18] -> M113/12(EB3)
  M113/1(LL1) -> Eval112/1(In1)
  M113/2(LL2) -> Eval112/2(In2)
  M113/3(LL3) -> Eval112/3(In3)
  Eval112/1(Out1) -> To Workspace112/1
  [in1] -> M114/1(CT1)
  [in5] -> M114/2(T1)
  [in6] -> M114/3(EB1)
  [in7] -> M114/4(CT2)
  [in8] -> M114/5(F2)
  [in9] -> M114/6(E2)
  [in10] -> M114/7(MR2)
  [in11] -> M114/8(T2)
  [in12] -> M114/9(EB2)
  [in13] -> M114/10(CT3)
  [in17] -> M114/11(T3)
  [in18] -> M114/12(EB3)
  M114/1(LL1) -> Eval113/1(In1)
  M114/2(LL2) -> Eval113/2(In2)
  M114/3(LL3) -> Eval113/3(In3)
  Eval113/1(Out1) -> To Workspace113/1
  [in1] -> M115/1(CT1)
  [in5] -> M115/2(T1)
  [in6] -> M115/3(EB1)
  [in7] -> M115/4(CT2)
  [in8] -> M115/5(F2)
  [in9] -> M115/6(E2)
  [in10] -> M115/7(MR2)
  [in11] -> M115/8(T2)
  [in12] -> M115/9(EB2)
  [in13] -> M115/10(CT3)
  [in17] -> M115/11(T3)
  [in18] -> M115/12(EB3)
  M115/1(LL1) -> Eval114/1(In1)
  M115/2(LL2) -> Eval114/2(In2)
  M115/3(LL3) -> Eval114/3(In3)
  Eval114/1(Out1) -> To Workspace114/1
  [in1] -> M116/1(CT1)
  [in5] -> M116/2(T1)
  [in6] -> M116/3(EB1)
  [in7] -> M116/4(CT2)
  [in8] -> M116/5(F2)
  [in9] -> M116/6(E2)
  [in10] -> M116/7(MR2)
  [in11] -> M116/8(T2)
  [in12] -> M116/9(EB2)
  [in13] -> M116/10(CT3)
  [in17] -> M116/11(T3)
  [in18] -> M116/12(EB3)
  M116/1(LL1) -> Eval115/1(In1)
  M116/2(LL2) -> Eval115/2(In2)
  M116/3(LL3) -> Eval115/3(In3)
  Eval115/1(Out1) -> To Workspace115/1
  [in1] -> M117/1(CT1)
  [in5] -> M117/2(T1)
  [in6] -> M117/3(EB1)
  [in7] -> M117/4(CT2)
  [in8] -> M117/5(F2)
  [in9] -> M117/6(E2)
  [in10] -> M117/7(MR2)
  [in11] -> M117/8(T2)
  [in12] -> M117/9(EB2)
  [in13] -> M117/10(CT3)
  [in17] -> M117/11(T3)
  [in18] -> M117/12(EB3)
  M117/1(LL1) -> Eval116/1(In1)
  M117/2(LL2) -> Eval116/2(In2)
  M117/3(LL3) -> Eval116/3(In3)
  Eval116/1(Out1) -> To Workspace116/1
  [in1] -> M118/1(CT1)
  [in5] -> M118/2(T1)
  [in6] -> M118/3(EB1)
  [in7] -> M118/4(CT2)
  [in8] -> M118/5(F2)
  [in9] -> M118/6(E2)
  [in10] -> M118/7(MR2)
  [in11] -> M118/8(T2)
  [in12] -> M118/9(EB2)
  [in13] -> M118/10(CT3)
  [in17] -> M118/11(T3)
  [in18] -> M118/12(EB3)
  M118/1(LL1) -> Eval117/1(In1)
  M118/2(LL2) -> Eval117/2(In2)
  M118/3(LL3) -> Eval117/3(In3)
  Eval117/1(Out1) -> To Workspace117/1
  [in1] -> M119/1(CT1)
  [in5] -> M119/2(T1)
  [in6] -> M119/3(EB1)
  [in7] -> M119/4(CT2)
  [in8] -> M119/5(F2)
  [in9] -> M119/6(E2)
  [in10] -> M119/7(MR2)
  [in11] -> M119/8(T2)
  [in12] -> M119/9(EB2)
  [in13] -> M119/10(CT3)
  [in17] -> M119/11(T3)
  [in18] -> M119/12(EB3)
  M119/1(LL1) -> Eval118/1(In1)
  M119/2(LL2) -> Eval118/2(In2)
  M119/3(LL3) -> Eval118/3(In3)
  Eval118/1(Out1) -> To Workspace118/1
  [in1] -> M120/1(CT1)
  [in5] -> M120/2(T1)
  [in6] -> M120/3(EB1)
  [in7] -> M120/4(CT2)
  [in8] -> M120/5(F2)
  [in9] -> M120/6(E2)
  [in10] -> M120/7(MR2)
  [in11] -> M120/8(T2)
  [in12] -> M120/9(EB2)
  [in13] -> M120/10(CT3)
  [in17] -> M120/11(T3)
  [in18] -> M120/12(EB3)
  M120/1(LL1) -> Eval119/1(In1)
  M120/2(LL2) -> Eval119/2(In2)
  M120/3(LL3) -> Eval119/3(In3)
  Eval119/1(Out1) -> To Workspace119/1
  [in1] -> M121/1(CT1)
  [in5] -> M121/2(T1)
  [in6] -> M121/3(EB1)
  [in7] -> M121/4(CT2)
  [in8] -> M121/5(F2)
  [in9] -> M121/6(E2)
  [in10] -> M121/7(MR2)
  [in11] -> M121/8(T2)
  [in12] -> M121/9(EB2)
  [in13] -> M121/10(CT3)
  [in17] -> M121/11(T3)
  [in18] -> M121/12(EB3)
  M121/1(LL1) -> Eval120/1(In1)
  M121/2(LL2) -> Eval120/2(In2)
  M121/3(LL3) -> Eval120/3(In3)
  Eval120/1(Out1) -> To Workspace120/1
  [in1] -> M122/1(CT1)
  [in5] -> M122/2(T1)
  [in6] -> M122/3(EB1)
  [in7] -> M122/4(CT2)
  [in8] -> M122/5(F2)
  [in9] -> M122/6(E2)
  [in10] -> M122/7(MR2)
  [in11] -> M122/8(T2)
  [in12] -> M122/9(EB2)
  [in13] -> M122/10(CT3)
  [in17] -> M122/11(T3)
  [in18] -> M122/12(EB3)
  M122/1(LL1) -> Eval121/1(In1)
  M122/2(LL2) -> Eval121/2(In2)
  M122/3(LL3) -> Eval121/3(In3)
  Eval121/1(Out1) -> To Workspace121/1
  [in1] -> M123/1(CT1)
  [in5] -> M123/2(T1)
  [in6] -> M123/3(EB1)
  [in7] -> M123/4(CT2)
  [in8] -> M123/5(F2)
  [in9] -> M123/6(E2)
  [in10] -> M123/7(MR2)
  [in11] -> M123/8(T2)
  [in12] -> M123/9(EB2)
  [in13] -> M123/10(CT3)
  [in17] -> M123/11(T3)
  [in18] -> M123/12(EB3)
  M123/1(LL1) -> Eval122/1(In1)
  M123/2(LL2) -> Eval122/2(In2)
  M123/3(LL3) -> Eval122/3(In3)
  Eval122/1(Out1) -> To Workspace122/1
  [in1] -> M124/1(CT1)
  [in5] -> M124/2(T1)
  [in6] -> M124/3(EB1)
  [in7] -> M124/4(CT2)
  [in8] -> M124/5(F2)
  [in9] -> M124/6(E2)
  [in10] -> M124/7(MR2)
  [in11] -> M124/8(T2)
  [in12] -> M124/9(EB2)
  [in13] -> M124/10(CT3)
  [in17] -> M124/11(T3)
  [in18] -> M124/12(EB3)
  M124/1(LL1) -> Eval123/1(In1)
  M124/2(LL2) -> Eval123/2(In2)
  M124/3(LL3) -> Eval123/3(In3)
  Eval123/1(Out1) -> To Workspace123/1
  [in1] -> M125/1(CT1)
  [in5] -> M125/2(T1)
  [in6] -> M125/3(EB1)
  [in7] -> M125/4(CT2)
  [in8] -> M125/5(F2)
  [in9] -> M125/6(E2)
  [in10] -> M125/7(MR2)
  [in11] -> M125/8(T2)
  [in12] -> M125/9(EB2)
  [in13] -> M125/10(CT3)
  [in17] -> M125/11(T3)
  [in18] -> M125/12(EB3)
  M125/1(LL1) -> Eval124/1(In1)
  M125/2(LL2) -> Eval124/2(In2)
  M125/3(LL3) -> Eval124/3(In3)
  Eval124/1(Out1) -> To Workspace124/1
  [in1] -> M126/1(CT1)
  [in5] -> M126/2(T1)
  [in6] -> M126/3(EB1)
  [in7] -> M126/4(CT2)
  [in8] -> M126/5(F2)
  [in9] -> M126/6(E2)
  [in10] -> M126/7(MR2)
  [in11] -> M126/8(T2)
  [in12] -> M126/9(EB2)
  [in13] -> M126/10(CT3)
  [in17] -> M126/11(T3)
  [in18] -> M126/12(EB3)
  M126/1(LL1) -> Eval125/1(In1)
  M126/2(LL2) -> Eval125/2(In2)
  M126/3(LL3) -> Eval125/3(In3)
  Eval125/1(Out1) -> To Workspace125/1
  [in1] -> M127/1(CT1)
  [in5] -> M127/2(T1)
  [in6] -> M127/3(EB1)
  [in7] -> M127/4(CT2)
  [in8] -> M127/5(F2)
  [in9] -> M127/6(E2)
  [in10] -> M127/7(MR2)
  [in11] -> M127/8(T2)
  [in12] -> M127/9(EB2)
  [in13] -> M127/10(CT3)
  [in17] -> M127/11(T3)
  [in18] -> M127/12(EB3)
  M127/1(LL1) -> Eval126/1(In1)
  M127/2(LL2) -> Eval126/2(In2)
  M127/3(LL3) -> Eval126/3(In3)
  Eval126/1(Out1) -> To Workspace126/1
  [in1] -> M128/1(CT1)
  [in5] -> M128/2(T1)
  [in6] -> M128/3(EB1)
  [in7] -> M128/4(CT2)
  [in8] -> M128/5(F2)
  [in9] -> M128/6(E2)
  [in10] -> M128/7(MR2)
  [in11] -> M128/8(T2)
  [in12] -> M128/9(EB2)
  [in13] -> M128/10(CT3)
  [in17] -> M128/11(T3)
  [in18] -> M128/12(EB3)
  M128/1(LL1) -> Eval127/1(In1)
  M128/2(LL2) -> Eval127/2(In2)
  M128/3(LL3) -> Eval127/3(In3)
  Eval127/1(Out1) -> To Workspace127/1
  [in1] -> M129/1(CT1)
  [in5] -> M129/2(T1)
  [in6] -> M129/3(EB1)
  [in7] -> M129/4(CT2)
  [in8] -> M129/5(F2)
  [in9] -> M129/6(E2)
  [in10] -> M129/7(MR2)
  [in11] -> M129/8(T2)
  [in12] -> M129/9(EB2)
  [in13] -> M129/10(CT3)
  [in17] -> M129/11(T3)
  [in18] -> M129/12(EB3)
  M129/1(LL1) -> Eval128/1(In1)
  M129/2(LL2) -> Eval128/2(In2)
  M129/3(LL3) -> Eval128/3(In3)
  Eval128/1(Out1) -> To Workspace128/1
  [in1] -> M130/1(CT1)
  [in5] -> M130/2(T1)
  [in6] -> M130/3(EB1)
  [in7] -> M130/4(CT2)
  [in8] -> M130/5(F2)
  [in9] -> M130/6(E2)
  [in10] -> M130/7(MR2)
  [in11] -> M130/8(T2)
  [in12] -> M130/9(EB2)
  [in13] -> M130/10(CT3)
  [in17] -> M130/11(T3)
  [in18] -> M130/12(EB3)
  M130/1(LL1) -> Eval129/1(In1)
  M130/2(LL2) -> Eval129/2(In2)
  M130/3(LL3) -> Eval129/3(In3)
  Eval129/1(Out1) -> To Workspace129/1
  [in1] -> M131/1(CT1)
  [in5] -> M131/2(T1)
  [in6] -> M131/3(EB1)
  [in7] -> M131/4(CT2)
  [in8] -> M131/5(F2)
  [in9] -> M131/6(E2)
  [in10] -> M131/7(MR2)
  [in11] -> M131/8(T2)
  [in12] -> M131/9(EB2)
  [in13] -> M131/10(CT3)
  [in17] -> M131/11(T3)
  [in18] -> M131/12(EB3)
  M131/1(LL1) -> Eval130/1(In1)
  M131/2(LL2) -> Eval130/2(In2)
  M131/3(LL3) -> Eval130/3(In3)
  Eval130/1(Out1) -> To Workspace130/1
  [in1] -> M132/1(CT1)
  [in5] -> M132/2(T1)
  [in6] -> M132/3(EB1)
  [in7] -> M132/4(CT2)
  [in8] -> M132/5(F2)
  [in9] -> M132/6(E2)
  [in10] -> M132/7(MR2)
  [in11] -> M132/8(T2)
  [in12] -> M132/9(EB2)
  [in13] -> M132/10(CT3)
  [in17] -> M132/11(T3)
  [in18] -> M132/12(EB3)
  M132/1(LL1) -> Eval131/1(In1)
  M132/2(LL2) -> Eval131/2(In2)
  M132/3(LL3) -> Eval131/3(In3)
  Eval131/1(Out1) -> To Workspace131/1
  [in1] -> M133/1(CT1)
  [in5] -> M133/2(T1)
  [in6] -> M133/3(EB1)
  [in7] -> M133/4(CT2)
  [in8] -> M133/5(F2)
  [in9] -> M133/6(E2)
  [in10] -> M133/7(MR2)
  [in11] -> M133/8(T2)
  [in12] -> M133/9(EB2)
  [in13] -> M133/10(CT3)
  [in17] -> M133/11(T3)
  [in18] -> M133/12(EB3)
  M133/1(LL1) -> Eval132/1(In1)
  M133/2(LL2) -> Eval132/2(In2)
  M133/3(LL3) -> Eval132/3(In3)
  Eval132/1(Out1) -> To Workspace132/1
  [in1] -> M134/1(CT1)
  [in5] -> M134/2(T1)
  [in6] -> M134/3(EB1)
  [in7] -> M134/4(CT2)
  [in8] -> M134/5(F2)
  [in9] -> M134/6(E2)
  [in10] -> M134/7(MR2)
  [in11] -> M134/8(T2)
  [in12] -> M134/9(EB2)
  [in13] -> M134/10(CT3)
  [in17] -> M134/11(T3)
  [in18] -> M134/12(EB3)
  M134/1(LL1) -> Eval133/1(In1)
  M134/2(LL2) -> Eval133/2(In2)
  M134/3(LL3) -> Eval133/3(In3)
  Eval133/1(Out1) -> To Workspace133/1
  [in1] -> M135/1(CT1)
  [in5] -> M135/2(T1)
  [in6] -> M135/3(EB1)
  [in7] -> M135/4(CT2)
  [in8] -> M135/5(F2)
  [in9] -> M135/6(E2)
  [in10] -> M135/7(MR2)
  [in11] -> M135/8(T2)
  [in12] -> M135/9(EB2)
  [in13] -> M135/10(CT3)
  [in17] -> M135/11(T3)
  [in18] -> M135/12(EB3)
  M135/1(LL1) -> Eval134/1(In1)
  M135/2(LL2) -> Eval134/2(In2)
  M135/3(LL3) -> Eval134/3(In3)
  Eval134/1(Out1) -> To Workspace134/1
  [in1] -> M136/1(CT1)
  [in5] -> M136/2(T1)
  [in6] -> M136/3(EB1)
  [in7] -> M136/4(CT2)
  [in8] -> M136/5(F2)
  [in9] -> M136/6(E2)
  [in10] -> M136/7(MR2)
  [in11] -> M136/8(T2)
  [in12] -> M136/9(EB2)
  [in13] -> M136/10(CT3)
  [in17] -> M136/11(T3)
  [in18] -> M136/12(EB3)
  M136/1(LL1) -> Eval135/1(In1)
  M136/2(LL2) -> Eval135/2(In2)
  M136/3(LL3) -> Eval135/3(In3)
  Eval135/1(Out1) -> To Workspace135/1
  [in1] -> M137/1(CT1)
  [in5] -> M137/2(T1)
  [in6] -> M137/3(EB1)
  [in7] -> M137/4(CT2)
  [in8] -> M137/5(F2)
  [in9] -> M137/6(E2)
  [in10] -> M137/7(MR2)
  [in11] -> M137/8(T2)
  [in12] -> M137/9(EB2)
  [in13] -> M137/10(CT3)
  [in17] -> M137/11(T3)
  [in18] -> M137/12(EB3)
  M137/1(LL1) -> Eval136/1(In1)
  M137/2(LL2) -> Eval136/2(In2)
  M137/3(LL3) -> Eval136/3(In3)
  Eval136/1(Out1) -> To Workspace136/1
  [in1] -> M138/1(CT1)
  [in5] -> M138/2(T1)
  [in6] -> M138/3(EB1)
  [in7] -> M138/4(CT2)
  [in8] -> M138/5(F2)
  [in9] -> M138/6(E2)
  [in10] -> M138/7(MR2)
  [in11] -> M138/8(T2)
  [in12] -> M138/9(EB2)
  [in13] -> M138/10(CT3)
  [in17] -> M138/11(T3)
  [in18] -> M138/12(EB3)
  M138/1(LL1) -> Eval137/1(In1)
  M138/2(LL2) -> Eval137/2(In2)
  M138/3(LL3) -> Eval137/3(In3)
  Eval137/1(Out1) -> To Workspace137/1
  [in1] -> M139/1(CT1)
  [in5] -> M139/2(T1)
  [in6] -> M139/3(EB1)
  [in7] -> M139/4(CT2)
  [in8] -> M139/5(F2)
  [in9] -> M139/6(E2)
  [in10] -> M139/7(MR2)
  [in11] -> M139/8(T2)
  [in12] -> M139/9(EB2)
  [in13] -> M139/10(CT3)
  [in17] -> M139/11(T3)
  [in18] -> M139/12(EB3)
  M139/1(LL1) -> Eval138/1(In1)
  M139/2(LL2) -> Eval138/2(In2)
  M139/3(LL3) -> Eval138/3(In3)
  Eval138/1(Out1) -> To Workspace138/1
  [in1] -> M140/1(CT1)
  [in5] -> M140/2(T1)
  [in6] -> M140/3(EB1)
  [in7] -> M140/4(CT2)
  [in8] -> M140/5(F2)
  [in9] -> M140/6(E2)
  [in10] -> M140/7(MR2)
  [in11] -> M140/8(T2)
  [in12] -> M140/9(EB2)
  [in13] -> M140/10(CT3)
  [in17] -> M140/11(T3)
  [in18] -> M140/12(EB3)
  M140/1(LL1) -> Eval139/1(In1)
  M140/2(LL2) -> Eval139/2(In2)
  M140/3(LL3) -> Eval139/3(In3)
  Eval139/1(Out1) -> To Workspace139/1
  [in1] -> M141/1(CT1)
  [in5] -> M141/2(T1)
  [in6] -> M141/3(EB1)
  [in7] -> M141/4(CT2)
  [in8] -> M141/5(F2)
  [in9] -> M141/6(E2)
  [in10] -> M141/7(MR2)
  [in11] -> M141/8(T2)
  [in12] -> M141/9(EB2)
  [in13] -> M141/10(CT3)
  [in17] -> M141/11(T3)
  [in18] -> M141/12(EB3)
  M141/1(LL1) -> Eval140/1(In1)
  M141/2(LL2) -> Eval140/2(In2)
  M141/3(LL3) -> Eval140/3(In3)
  Eval140/1(Out1) -> To Workspace140/1
  [in1] -> M142/1(CT1)
  [in5] -> M142/2(T1)
  [in6] -> M142/3(EB1)
  [in7] -> M142/4(CT2)
  [in8] -> M142/5(F2)
  [in9] -> M142/6(E2)
  [in10] -> M142/7(MR2)
  [in11] -> M142/8(T2)
  [in12] -> M142/9(EB2)
  [in13] -> M142/10(CT3)
  [in17] -> M142/11(T3)
  [in18] -> M142/12(EB3)
  M142/1(LL1) -> Eval141/1(In1)
  M142/2(LL2) -> Eval141/2(In2)
  M142/3(LL3) -> Eval141/3(In3)
  Eval141/1(Out1) -> To Workspace141/1
  [in1] -> M143/1(CT1)
  [in5] -> M143/2(T1)
  [in6] -> M143/3(EB1)
  [in7] -> M143/4(CT2)
  [in8] -> M143/5(F2)
  [in9] -> M143/6(E2)
  [in10] -> M143/7(MR2)
  [in11] -> M143/8(T2)
  [in12] -> M143/9(EB2)
  [in13] -> M143/10(CT3)
  [in17] -> M143/11(T3)
  [in18] -> M143/12(EB3)
  M143/1(LL1) -> Eval142/1(In1)
  M143/2(LL2) -> Eval142/2(In2)
  M143/3(LL3) -> Eval142/3(In3)
  Eval142/1(Out1) -> To Workspace142/1
  [in1] -> M144/1(CT1)
  [in5] -> M144/2(T1)
  [in6] -> M144/3(EB1)
  [in7] -> M144/4(CT2)
  [in8] -> M144/5(F2)
  [in9] -> M144/6(E2)
  [in10] -> M144/7(MR2)
  [in11] -> M144/8(T2)
  [in12] -> M144/9(EB2)
  [in13] -> M144/10(CT3)
  [in17] -> M144/11(T3)
  [in18] -> M144/12(EB3)
  M144/1(LL1) -> Eval143/1(In1)
  M144/2(LL2) -> Eval143/2(In2)
  M144/3(LL3) -> Eval143/3(In3)
  Eval143/1(Out1) -> To Workspace143/1
  [in1] -> M145/1(CT1)
  [in5] -> M145/2(T1)
  [in6] -> M145/3(EB1)
  [in7] -> M145/4(CT2)
  [in8] -> M145/5(F2)
  [in9] -> M145/6(E2)
  [in10] -> M145/7(MR2)
  [in11] -> M145/8(T2)
  [in12] -> M145/9(EB2)
  [in13] -> M145/10(CT3)
  [in17] -> M145/11(T3)
  [in18] -> M145/12(EB3)
  M145/1(LL1) -> Eval144/1(In1)
  M145/2(LL2) -> Eval144/2(In2)
  M145/3(LL3) -> Eval144/3(In3)
  Eval144/1(Out1) -> To Workspace144/1
  [in1] -> M146/1(CT1)
  [in5] -> M146/2(T1)
  [in6] -> M146/3(EB1)
  [in7] -> M146/4(CT2)
  [in8] -> M146/5(F2)
  [in9] -> M146/6(E2)
  [in10] -> M146/7(MR2)
  [in11] -> M146/8(T2)
  [in12] -> M146/9(EB2)
  [in13] -> M146/10(CT3)
  [in17] -> M146/11(T3)
  [in18] -> M146/12(EB3)
  M146/1(LL1) -> Eval145/1(In1)
  M146/2(LL2) -> Eval145/2(In2)
  M146/3(LL3) -> Eval145/3(In3)
  Eval145/1(Out1) -> To Workspace145/1
  [in1] -> M147/1(CT1)
  [in5] -> M147/2(T1)
  [in6] -> M147/3(EB1)
  [in7] -> M147/4(CT2)
  [in8] -> M147/5(F2)
  [in9] -> M147/6(E2)
  [in10] -> M147/7(MR2)
  [in11] -> M147/8(T2)
  [in12] -> M147/9(EB2)
  [in13] -> M147/10(CT3)
  [in17] -> M147/11(T3)
  [in18] -> M147/12(EB3)
  M147/1(LL1) -> Eval146/1(In1)
  M147/2(LL2) -> Eval146/2(In2)
  M147/3(LL3) -> Eval146/3(In3)
  Eval146/1(Out1) -> To Workspace146/1
  [in1] -> M148/1(CT1)
  [in5] -> M148/2(T1)
  [in6] -> M148/3(EB1)
  [in7] -> M148/4(CT2)
  [in8] -> M148/5(F2)
  [in9] -> M148/6(E2)
  [in10] -> M148/7(MR2)
  [in11] -> M148/8(T2)
  [in12] -> M148/9(EB2)
  [in13] -> M148/10(CT3)
  [in17] -> M148/11(T3)
  [in18] -> M148/12(EB3)
  M148/1(LL1) -> Eval147/1(In1)
  M148/2(LL2) -> Eval147/2(In2)
  M148/3(LL3) -> Eval147/3(In3)
  Eval147/1(Out1) -> To Workspace147/1
  [in1] -> M149/1(CT1)
  [in5] -> M149/2(T1)
  [in6] -> M149/3(EB1)
  [in7] -> M149/4(CT2)
  [in8] -> M149/5(F2)
  [in9] -> M149/6(E2)
  [in10] -> M149/7(MR2)
  [in11] -> M149/8(T2)
  [in12] -> M149/9(EB2)
  [in13] -> M149/10(CT3)
  [in17] -> M149/11(T3)
  [in18] -> M149/12(EB3)
  M149/1(LL1) -> Eval148/1(In1)
  M149/2(LL2) -> Eval148/2(In2)
  M149/3(LL3) -> Eval148/3(In3)
  Eval148/1(Out1) -> To Workspace148/1
  [in1] -> M150/1(CT1)
  [in5] -> M150/2(T1)
  [in6] -> M150/3(EB1)
  [in7] -> M150/4(CT2)
  [in8] -> M150/5(F2)
  [in9] -> M150/6(E2)
  [in10] -> M150/7(MR2)
  [in11] -> M150/8(T2)
  [in12] -> M150/9(EB2)
  [in13] -> M150/10(CT3)
  [in17] -> M150/11(T3)
  [in18] -> M150/12(EB3)
  M150/1(LL1) -> Eval149/1(In1)
  M150/2(LL2) -> Eval149/2(In2)
  M150/3(LL3) -> Eval149/3(In3)
  Eval149/1(Out1) -> To Workspace149/1
  [in1] -> M151/1(CT1)
  [in5] -> M151/2(T1)
  [in6] -> M151/3(EB1)
  [in7] -> M151/4(CT2)
  [in8] -> M151/5(F2)
  [in9] -> M151/6(E2)
  [in10] -> M151/7(MR2)
  [in11] -> M151/8(T2)
  [in12] -> M151/9(EB2)
  [in13] -> M151/10(CT3)
  [in17] -> M151/11(T3)
  [in18] -> M151/12(EB3)
  M151/1(LL1) -> Eval150/1(In1)
  M151/2(LL2) -> Eval150/2(In2)
  M151/3(LL3) -> Eval150/3(In3)
  Eval150/1(Out1) -> To Workspace150/1
  [in1] -> M152/1(CT1)
  [in5] -> M152/2(T1)
  [in6] -> M152/3(EB1)
  [in7] -> M152/4(CT2)
  [in8] -> M152/5(F2)
  [in9] -> M152/6(E2)
  [in10] -> M152/7(MR2)
  [in11] -> M152/8(T2)
  [in12] -> M152/9(EB2)
  [in13] -> M152/10(CT3)
  [in17] -> M152/11(T3)
  [in18] -> M152/12(EB3)
  M152/1(LL1) -> Eval151/1(In1)
  M152/2(LL2) -> Eval151/2(In2)
  M152/3(LL3) -> Eval151/3(In3)
  Eval151/1(Out1) -> To Workspace151/1
  [in1] -> M153/1(CT1)
  [in5] -> M153/2(T1)
  [in6] -> M153/3(EB1)
  [in7] -> M153/4(CT2)
  [in8] -> M153/5(F2)
  [in9] -> M153/6(E2)
  [in10] -> M153/7(MR2)
  [in11] -> M153/8(T2)
  [in12] -> M153/9(EB2)
  [in13] -> M153/10(CT3)
  [in17] -> M153/11(T3)
  [in18] -> M153/12(EB3)
  M153/1(LL1) -> Eval152/1(In1)
  M153/2(LL2) -> Eval152/2(In2)
  M153/3(LL3) -> Eval152/3(In3)
  Eval152/1(Out1) -> To Workspace152/1
  [in1] -> M154/1(CT1)
  [in5] -> M154/2(T1)
  [in6] -> M154/3(EB1)
  [in7] -> M154/4(CT2)
  [in8] -> M154/5(F2)
  [in9] -> M154/6(E2)
  [in10] -> M154/7(MR2)
  [in11] -> M154/8(T2)
  [in12] -> M154/9(EB2)
  [in13] -> M154/10(CT3)
  [in17] -> M154/11(T3)
  [in18] -> M154/12(EB3)
  M154/1(LL1) -> Eval153/1(In1)
  M154/2(LL2) -> Eval153/2(In2)
  M154/3(LL3) -> Eval153/3(In3)
  Eval153/1(Out1) -> To Workspace153/1
  [in1] -> M155/1(CT1)
  [in5] -> M155/2(T1)
  [in6] -> M155/3(EB1)
  [in7] -> M155/4(CT2)
  [in8] -> M155/5(F2)
  [in9] -> M155/6(E2)
  [in10] -> M155/7(MR2)
  [in11] -> M155/8(T2)
  [in12] -> M155/9(EB2)
  [in13] -> M155/10(CT3)
  [in17] -> M155/11(T3)
  [in18] -> M155/12(EB3)
  M155/1(LL1) -> Eval154/1(In1)
  M155/2(LL2) -> Eval154/2(In2)
  M155/3(LL3) -> Eval154/3(In3)
  Eval154/1(Out1) -> To Workspace154/1
  [in1] -> M156/1(CT1)
  [in5] -> M156/2(T1)
  [in6] -> M156/3(EB1)
  [in7] -> M156/4(CT2)
  [in8] -> M156/5(F2)
  [in9] -> M156/6(E2)
  [in10] -> M156/7(MR2)
  [in11] -> M156/8(T2)
  [in12] -> M156/9(EB2)
  [in13] -> M156/10(CT3)
  [in17] -> M156/11(T3)
  [in18] -> M156/12(EB3)
  M156/1(LL1) -> Eval155/1(In1)
  M156/2(LL2) -> Eval155/2(In2)
  M156/3(LL3) -> Eval155/3(In3)
  Eval155/1(Out1) -> To Workspace155/1
  [in1] -> M157/1(CT1)
  [in5] -> M157/2(T1)
  [in6] -> M157/3(EB1)
  [in7] -> M157/4(CT2)
  [in8] -> M157/5(F2)
  [in9] -> M157/6(E2)
  [in10] -> M157/7(MR2)
  [in11] -> M157/8(T2)
  [in12] -> M157/9(EB2)
  [in13] -> M157/10(CT3)
  [in17] -> M157/11(T3)
  [in18] -> M157/12(EB3)
  M157/1(LL1) -> Eval156/1(In1)
  M157/2(LL2) -> Eval156/2(In2)
  M157/3(LL3) -> Eval156/3(In3)
  Eval156/1(Out1) -> To Workspace156/1
  [in1] -> M158/1(CT1)
  [in5] -> M158/2(T1)
  [in6] -> M158/3(EB1)
  [in7] -> M158/4(CT2)
  [in8] -> M158/5(F2)
  [in9] -> M158/6(E2)
  [in10] -> M158/7(MR2)
  [in11] -> M158/8(T2)
  [in12] -> M158/9(EB2)
  [in13] -> M158/10(CT3)
  [in17] -> M158/11(T3)
  [in18] -> M158/12(EB3)
  M158/1(LL1) -> Eval157/1(In1)
  M158/2(LL2) -> Eval157/2(In2)
  M158/3(LL3) -> Eval157/3(In3)
  Eval157/1(Out1) -> To Workspace157/1
  [in1] -> M159/1(CT1)
  [in5] -> M159/2(T1)
  [in6] -> M159/3(EB1)
  [in7] -> M159/4(CT2)
  [in8] -> M159/5(F2)
  [in9] -> M159/6(E2)
  [in10] -> M159/7(MR2)
  [in11] -> M159/8(T2)
  [in12] -> M159/9(EB2)
  [in13] -> M159/10(CT3)
  [in17] -> M159/11(T3)
  [in18] -> M159/12(EB3)
  M159/1(LL1) -> Eval158/1(In1)
  M159/2(LL2) -> Eval158/2(In2)
  M159/3(LL3) -> Eval158/3(In3)
  Eval158/1(Out1) -> To Workspace158/1
  [in1] -> M160/1(CT1)
  [in5] -> M160/2(T1)
  [in6] -> M160/3(EB1)
  [in7] -> M160/4(CT2)
  [in8] -> M160/5(F2)
  [in9] -> M160/6(E2)
  [in10] -> M160/7(MR2)
  [in11] -> M160/8(T2)
  [in12] -> M160/9(EB2)
  [in13] -> M160/10(CT3)
  [in17] -> M160/11(T3)
  [in18] -> M160/12(EB3)
  M160/1(LL1) -> Eval159/1(In1)
  M160/2(LL2) -> Eval159/2(In2)
  M160/3(LL3) -> Eval159/3(In3)
  Eval159/1(Out1) -> To Workspace159/1
  [in1] -> M161/1(CT1)
  [in5] -> M161/2(T1)
  [in6] -> M161/3(EB1)
  [in7] -> M161/4(CT2)
  [in8] -> M161/5(F2)
  [in9] -> M161/6(E2)
  [in10] -> M161/7(MR2)
  [in11] -> M161/8(T2)
  [in12] -> M161/9(EB2)
  [in13] -> M161/10(CT3)
  [in17] -> M161/11(T3)
  [in18] -> M161/12(EB3)
  M161/1(LL1) -> Eval160/1(In1)
  M161/2(LL2) -> Eval160/2(In2)
  M161/3(LL3) -> Eval160/3(In3)
  Eval160/1(Out1) -> To Workspace160/1
  [in1] -> M162/1(CT1)
  [in5] -> M162/2(T1)
  [in6] -> M162/3(EB1)
  [in7] -> M162/4(CT2)
  [in8] -> M162/5(F2)
  [in9] -> M162/6(E2)
  [in10] -> M162/7(MR2)
  [in11] -> M162/8(T2)
  [in12] -> M162/9(EB2)
  [in13] -> M162/10(CT3)
  [in17] -> M162/11(T3)
  [in18] -> M162/12(EB3)
  M162/1(LL1) -> Eval161/1(In1)
  M162/2(LL2) -> Eval161/2(In2)
  M162/3(LL3) -> Eval161/3(In3)
  Eval161/1(Out1) -> To Workspace161/1
  [in1] -> M163/1(CT1)
  [in5] -> M163/2(T1)
  [in6] -> M163/3(EB1)
  [in7] -> M163/4(CT2)
  [in8] -> M163/5(F2)
  [in9] -> M163/6(E2)
  [in10] -> M163/7(MR2)
  [in11] -> M163/8(T2)
  [in12] -> M163/9(EB2)
  [in13] -> M163/10(CT3)
  [in17] -> M163/11(T3)
  [in18] -> M163/12(EB3)
  M163/1(LL1) -> Eval162/1(In1)
  M163/2(LL2) -> Eval162/2(In2)
  M163/3(LL3) -> Eval162/3(In3)
  Eval162/1(Out1) -> To Workspace162/1
  [in1] -> M164/1(CT1)
  [in5] -> M164/2(T1)
  [in6] -> M164/3(EB1)
  [in7] -> M164/4(CT2)
  [in8] -> M164/5(F2)
  [in9] -> M164/6(E2)
  [in10] -> M164/7(MR2)
  [in11] -> M164/8(T2)
  [in12] -> M164/9(EB2)
  [in13] -> M164/10(CT3)
  [in17] -> M164/11(T3)
  [in18] -> M164/12(EB3)
  M164/1(LL1) -> Eval163/1(In1)
  M164/2(LL2) -> Eval163/2(In2)
  M164/3(LL3) -> Eval163/3(In3)
  Eval163/1(Out1) -> To Workspace163/1
  [in1] -> M165/1(CT1)
  [in5] -> M165/2(T1)
  [in6] -> M165/3(EB1)
  [in7] -> M165/4(CT2)
  [in8] -> M165/5(F2)
  [in9] -> M165/6(E2)
  [in10] -> M165/7(MR2)
  [in11] -> M165/8(T2)
  [in12] -> M165/9(EB2)
  [in13] -> M165/10(CT3)
  [in17] -> M165/11(T3)
  [in18] -> M165/12(EB3)
  M165/1(LL1) -> Eval164/1(In1)
  M165/2(LL2) -> Eval164/2(In2)
  M165/3(LL3) -> Eval164/3(In3)
  Eval164/1(Out1) -> To Workspace164/1
  [in1] -> M166/1(CT1)
  [in5] -> M166/2(T1)
  [in6] -> M166/3(EB1)
  [in7] -> M166/4(CT2)
  [in8] -> M166/5(F2)
  [in9] -> M166/6(E2)
  [in10] -> M166/7(MR2)
  [in11] -> M166/8(T2)
  [in12] -> M166/9(EB2)
  [in13] -> M166/10(CT3)
  [in17] -> M166/11(T3)
  [in18] -> M166/12(EB3)
  M166/1(LL1) -> Eval165/1(In1)
  M166/2(LL2) -> Eval165/2(In2)
  M166/3(LL3) -> Eval165/3(In3)
  Eval165/1(Out1) -> To Workspace165/1
  [in1] -> M167/1(CT1)
  [in5] -> M167/2(T1)
  [in6] -> M167/3(EB1)
  [in7] -> M167/4(CT2)
  [in8] -> M167/5(F2)
  [in9] -> M167/6(E2)
  [in10] -> M167/7(MR2)
  [in11] -> M167/8(T2)
  [in12] -> M167/9(EB2)
  [in13] -> M167/10(CT3)
  [in17] -> M167/11(T3)
  [in18] -> M167/12(EB3)
  M167/1(LL1) -> Eval166/1(In1)
  M167/2(LL2) -> Eval166/2(In2)
  M167/3(LL3) -> Eval166/3(In3)
  Eval166/1(Out1) -> To Workspace166/1
  [in1] -> M168/1(CT1)
  [in5] -> M168/2(T1)
  [in6] -> M168/3(EB1)
  [in7] -> M168/4(CT2)
  [in8] -> M168/5(F2)
  [in9] -> M168/6(E2)
  [in10] -> M168/7(MR2)
  [in11] -> M168/8(T2)
  [in12] -> M168/9(EB2)
  [in13] -> M168/10(CT3)
  [in17] -> M168/11(T3)
  [in18] -> M168/12(EB3)
  M168/1(LL1) -> Eval167/1(In1)
  M168/2(LL2) -> Eval167/2(In2)
  M168/3(LL3) -> Eval167/3(In3)
  Eval167/1(Out1) -> To Workspace167/1
  [in1] -> M169/1(CT1)
  [in5] -> M169/2(T1)
  [in6] -> M169/3(EB1)
  [in7] -> M169/4(CT2)
  [in8] -> M169/5(F2)
  [in9] -> M169/6(E2)
  [in10] -> M169/7(MR2)
  [in11] -> M169/8(T2)
  [in12] -> M169/9(EB2)
  [in13] -> M169/10(CT3)
  [in17] -> M169/11(T3)
  [in18] -> M169/12(EB3)
  M169/1(LL1) -> Eval168/1(In1)
  M169/2(LL2) -> Eval168/2(In2)
  M169/3(LL3) -> Eval168/3(In3)
  Eval168/1(Out1) -> To Workspace168/1
  [in1] -> M170/1(CT1)
  [in5] -> M170/2(T1)
  [in6] -> M170/3(EB1)
  [in7] -> M170/4(CT2)
  [in8] -> M170/5(F2)
  [in9] -> M170/6(E2)
  [in10] -> M170/7(MR2)
  [in11] -> M170/8(T2)
  [in12] -> M170/9(EB2)
  [in13] -> M170/10(CT3)
  [in17] -> M170/11(T3)
  [in18] -> M170/12(EB3)
  M170/1(LL1) -> Eval169/1(In1)
  M170/2(LL2) -> Eval169/2(In2)
  M170/3(LL3) -> Eval169/3(In3)
  Eval169/1(Out1) -> To Workspace169/1
  [in1] -> M171/1(CT1)
  [in5] -> M171/2(T1)
  [in6] -> M171/3(EB1)
  [in7] -> M171/4(CT2)
  [in8] -> M171/5(F2)
  [in9] -> M171/6(E2)
  [in10] -> M171/7(MR2)
  [in11] -> M171/8(T2)
  [in12] -> M171/9(EB2)
  [in13] -> M171/10(CT3)
  [in17] -> M171/11(T3)
  [in18] -> M171/12(EB3)
  M171/1(LL1) -> Eval170/1(In1)
  M171/2(LL2) -> Eval170/2(In2)
  M171/3(LL3) -> Eval170/3(In3)
  Eval170/1(Out1) -> To Workspace170/1
  [in1] -> M172/1(CT1)
  [in5] -> M172/2(T1)
  [in6] -> M172/3(EB1)
  [in7] -> M172/4(CT2)
  [in8] -> M172/5(F2)
  [in9] -> M172/6(E2)
  [in10] -> M172/7(MR2)
  [in11] -> M172/8(T2)
  [in12] -> M172/9(EB2)
  [in13] -> M172/10(CT3)
  [in17] -> M172/11(T3)
  [in18] -> M172/12(EB3)
  M172/1(LL1) -> Eval171/1(In1)
  M172/2(LL2) -> Eval171/2(In2)
  M172/3(LL3) -> Eval171/3(In3)
  Eval171/1(Out1) -> To Workspace171/1
  [in1] -> M173/1(CT1)
  [in5] -> M173/2(T1)
  [in6] -> M173/3(EB1)
  [in7] -> M173/4(CT2)
  [in8] -> M173/5(F2)
  [in9] -> M173/6(E2)
  [in10] -> M173/7(MR2)
  [in11] -> M173/8(T2)
  [in12] -> M173/9(EB2)
  [in13] -> M173/10(CT3)
  [in17] -> M173/11(T3)
  [in18] -> M173/12(EB3)
  M173/1(LL1) -> Eval172/1(In1)
  M173/2(LL2) -> Eval172/2(In2)
  M173/3(LL3) -> Eval172/3(In3)
  Eval172/1(Out1) -> To Workspace172/1
  [in1] -> M174/1(CT1)
  [in5] -> M174/2(T1)
  [in6] -> M174/3(EB1)
  [in7] -> M174/4(CT2)
  [in8] -> M174/5(F2)
  [in9] -> M174/6(E2)
  [in10] -> M174/7(MR2)
  [in11] -> M174/8(T2)
  [in12] -> M174/9(EB2)
  [in13] -> M174/10(CT3)
  [in17] -> M174/11(T3)
  [in18] -> M174/12(EB3)
  M174/1(LL1) -> Eval173/1(In1)
  M174/2(LL2) -> Eval173/2(In2)
  M174/3(LL3) -> Eval173/3(In3)
  Eval173/1(Out1) -> To Workspace173/1
  [in1] -> M175/1(CT1)
  [in5] -> M175/2(T1)
  [in6] -> M175/3(EB1)
  [in7] -> M175/4(CT2)
  [in8] -> M175/5(F2)
  [in9] -> M175/6(E2)
  [in10] -> M175/7(MR2)
  [in11] -> M175/8(T2)
  [in12] -> M175/9(EB2)
  [in13] -> M175/10(CT3)
  [in17] -> M175/11(T3)
  [in18] -> M175/12(EB3)
  M175/1(LL1) -> Eval174/1(In1)
  M175/2(LL2) -> Eval174/2(In2)
  M175/3(LL3) -> Eval174/3(In3)
  Eval174/1(Out1) -> To Workspace174/1
  [in1] -> M176/1(CT1)
  [in5] -> M176/2(T1)
  [in6] -> M176/3(EB1)
  [in7] -> M176/4(CT2)
  [in8] -> M176/5(F2)
  [in9] -> M176/6(E2)
  [in10] -> M176/7(MR2)
  [in11] -> M176/8(T2)
  [in12] -> M176/9(EB2)
  [in13] -> M176/10(CT3)
  [in17] -> M176/11(T3)
  [in18] -> M176/12(EB3)
  M176/1(LL1) -> Eval175/1(In1)
  M176/2(LL2) -> Eval175/2(In2)
  M176/3(LL3) -> Eval175/3(In3)
  Eval175/1(Out1) -> To Workspace175/1
  [in1] -> M177/1(CT1)
  [in5] -> M177/2(T1)
  [in6] -> M177/3(EB1)
  [in7] -> M177/4(CT2)
  [in8] -> M177/5(F2)
  [in9] -> M177/6(E2)
  [in10] -> M177/7(MR2)
  [in11] -> M177/8(T2)
  [in12] -> M177/9(EB2)
  [in13] -> M177/10(CT3)
  [in17] -> M177/11(T3)
  [in18] -> M177/12(EB3)
  M177/1(LL1) -> Eval176/1(In1)
  M177/2(LL2) -> Eval176/2(In2)
  M177/3(LL3) -> Eval176/3(In3)
  Eval176/1(Out1) -> To Workspace176/1
  [in1] -> M178/1(CT1)
  [in5] -> M178/2(T1)
  [in6] -> M178/3(EB1)
  [in7] -> M178/4(CT2)
  [in8] -> M178/5(F2)
  [in9] -> M178/6(E2)
  [in10] -> M178/7(MR2)
  [in11] -> M178/8(T2)
  [in12] -> M178/9(EB2)
  [in13] -> M178/10(CT3)
  [in17] -> M178/11(T3)
  [in18] -> M178/12(EB3)
  M178/1(LL1) -> Eval177/1(In1)
  M178/2(LL2) -> Eval177/2(In2)
  M178/3(LL3) -> Eval177/3(In3)
  Eval177/1(Out1) -> To Workspace177/1
  [in1] -> M179/1(CT1)
  [in5] -> M179/2(T1)
  [in6] -> M179/3(EB1)
  [in7] -> M179/4(CT2)
  [in8] -> M179/5(F2)
  [in9] -> M179/6(E2)
  [in10] -> M179/7(MR2)
  [in11] -> M179/8(T2)
  [in12] -> M179/9(EB2)
  [in13] -> M179/10(CT3)
  [in17] -> M179/11(T3)
  [in18] -> M179/12(EB3)
  M179/1(LL1) -> Eval178/1(In1)
  M179/2(LL2) -> Eval178/2(In2)
  M179/3(LL3) -> Eval178/3(In3)
  Eval178/1(Out1) -> To Workspace178/1
  [in1] -> M180/1(CT1)
  [in5] -> M180/2(T1)
  [in6] -> M180/3(EB1)
  [in7] -> M180/4(CT2)
  [in8] -> M180/5(F2)
  [in9] -> M180/6(E2)
  [in10] -> M180/7(MR2)
  [in11] -> M180/8(T2)
  [in12] -> M180/9(EB2)
  [in13] -> M180/10(CT3)
  [in17] -> M180/11(T3)
  [in18] -> M180/12(EB3)
  M180/1(LL1) -> Eval179/1(In1)
  M180/2(LL2) -> Eval179/2(In2)
  M180/3(LL3) -> Eval179/3(In3)
  Eval179/1(Out1) -> To Workspace179/1
  [in1] -> M181/1(CT1)
  [in5] -> M181/2(T1)
  [in6] -> M181/3(EB1)
  [in7] -> M181/4(CT2)
  [in8] -> M181/5(F2)
  [in9] -> M181/6(E2)
  [in10] -> M181/7(MR2)
  [in11] -> M181/8(T2)
  [in12] -> M181/9(EB2)
  [in13] -> M181/10(CT3)
  [in17] -> M181/11(T3)
  [in18] -> M181/12(EB3)
  M181/1(LL1) -> Eval180/1(In1)
  M181/2(LL2) -> Eval180/2(In2)
  M181/3(LL3) -> Eval180/3(In3)
  Eval180/1(Out1) -> To Workspace180/1
  [in1] -> M182/1(CT1)
  [in5] -> M182/2(T1)
  [in6] -> M182/3(EB1)
  [in7] -> M182/4(CT2)
  [in8] -> M182/5(F2)
  [in9] -> M182/6(E2)
  [in10] -> M182/7(MR2)
  [in11] -> M182/8(T2)
  [in12] -> M182/9(EB2)
  [in13] -> M182/10(CT3)
  [in17] -> M182/11(T3)
  [in18] -> M182/12(EB3)
  M182/1(LL1) -> Eval181/1(In1)
  M182/2(LL2) -> Eval181/2(In2)
  M182/3(LL3) -> Eval181/3(In3)
  Eval181/1(Out1) -> To Workspace181/1
  [in1] -> M183/1(CT1)
  [in5] -> M183/2(T1)
  [in6] -> M183/3(EB1)
  [in7] -> M183/4(CT2)
  [in8] -> M183/5(F2)
  [in9] -> M183/6(E2)
  [in10] -> M183/7(MR2)
  [in11] -> M183/8(T2)
  [in12] -> M183/9(EB2)
  [in13] -> M183/10(CT3)
  [in17] -> M183/11(T3)
  [in18] -> M183/12(EB3)
  M183/1(LL1) -> Eval182/1(In1)
  M183/2(LL2) -> Eval182/2(In2)
  M183/3(LL3) -> Eval182/3(In3)
  Eval182/1(Out1) -> To Workspace182/1
  [in1] -> M184/1(CT1)
  [in5] -> M184/2(T1)
  [in6] -> M184/3(EB1)
  [in7] -> M184/4(CT2)
  [in8] -> M184/5(F2)
  [in9] -> M184/6(E2)
  [in10] -> M184/7(MR2)
  [in11] -> M184/8(T2)
  [in12] -> M184/9(EB2)
  [in13] -> M184/10(CT3)
  [in17] -> M184/11(T3)
  [in18] -> M184/12(EB3)
  M184/1(LL1) -> Eval183/1(In1)
  M184/2(LL2) -> Eval183/2(In2)
  M184/3(LL3) -> Eval183/3(In3)
  Eval183/1(Out1) -> To Workspace183/1
  [in1] -> M185/1(CT1)
  [in5] -> M185/2(T1)
  [in6] -> M185/3(EB1)
  [in7] -> M185/4(CT2)
  [in8] -> M185/5(F2)
  [in9] -> M185/6(E2)
  [in10] -> M185/7(MR2)
  [in11] -> M185/8(T2)
  [in12] -> M185/9(EB2)
  [in13] -> M185/10(CT3)
  [in17] -> M185/11(T3)
  [in18] -> M185/12(EB3)
  M185/1(LL1) -> Eval184/1(In1)
  M185/2(LL2) -> Eval184/2(In2)
  M185/3(LL3) -> Eval184/3(In3)
  Eval184/1(Out1) -> To Workspace184/1
  [in1] -> M186/1(CT1)
  [in5] -> M186/2(T1)
  [in6] -> M186/3(EB1)
  [in7] -> M186/4(CT2)
  [in8] -> M186/5(F2)
  [in9] -> M186/6(E2)
  [in10] -> M186/7(MR2)
  [in11] -> M186/8(T2)
  [in12] -> M186/9(EB2)
  [in13] -> M186/10(CT3)
  [in17] -> M186/11(T3)
  [in18] -> M186/12(EB3)
  M186/1(LL1) -> Eval185/1(In1)
  M186/2(LL2) -> Eval185/2(In2)
  M186/3(LL3) -> Eval185/3(In3)
  Eval185/1(Out1) -> To Workspace185/1
  [in1] -> M187/1(CT1)
  [in5] -> M187/2(T1)
  [in6] -> M187/3(EB1)
  [in7] -> M187/4(CT2)
  [in8] -> M187/5(F2)
  [in9] -> M187/6(E2)
  [in10] -> M187/7(MR2)
  [in11] -> M187/8(T2)
  [in12] -> M187/9(EB2)
  [in13] -> M187/10(CT3)
  [in17] -> M187/11(T3)
  [in18] -> M187/12(EB3)
  M187/1(LL1) -> Eval186/1(In1)
  M187/2(LL2) -> Eval186/2(In2)
  M187/3(LL3) -> Eval186/3(In3)
  Eval186/1(Out1) -> To Workspace186/1
  [in1] -> M188/1(CT1)
  [in5] -> M188/2(T1)
  [in6] -> M188/3(EB1)
  [in7] -> M188/4(CT2)
  [in8] -> M188/5(F2)
  [in9] -> M188/6(E2)
  [in10] -> M188/7(MR2)
  [in11] -> M188/8(T2)
  [in12] -> M188/9(EB2)
  [in13] -> M188/10(CT3)
  [in17] -> M188/11(T3)
  [in18] -> M188/12(EB3)
  M188/1(LL1) -> Eval187/1(In1)
  M188/2(LL2) -> Eval187/2(In2)
  M188/3(LL3) -> Eval187/3(In3)
  Eval187/1(Out1) -> To Workspace187/1
  [in1] -> M189/1(CT1)
  [in5] -> M189/2(T1)
  [in6] -> M189/3(EB1)
  [in7] -> M189/4(CT2)
  [in8] -> M189/5(F2)
  [in9] -> M189/6(E2)
  [in10] -> M189/7(MR2)
  [in11] -> M189/8(T2)
  [in12] -> M189/9(EB2)
  [in13] -> M189/10(CT3)
  [in17] -> M189/11(T3)
  [in18] -> M189/12(EB3)
  M189/1(LL1) -> Eval188/1(In1)
  M189/2(LL2) -> Eval188/2(In2)
  M189/3(LL3) -> Eval188/3(In3)
  Eval188/1(Out1) -> To Workspace188/1
  [in1] -> M190/1(CT1)
  [in5] -> M190/2(T1)
  [in6] -> M190/3(EB1)
  [in7] -> M190/4(CT2)
  [in8] -> M190/5(F2)
  [in9] -> M190/6(E2)
  [in10] -> M190/7(MR2)
  [in11] -> M190/8(T2)
  [in12] -> M190/9(EB2)
  [in13] -> M190/10(CT3)
  [in17] -> M190/11(T3)
  [in18] -> M190/12(EB3)
  M190/1(LL1) -> Eval189/1(In1)
  M190/2(LL2) -> Eval189/2(In2)
  M190/3(LL3) -> Eval189/3(In3)
  Eval189/1(Out1) -> To Workspace189/1
  [in1] -> M191/1(CT1)
  [in5] -> M191/2(T1)
  [in6] -> M191/3(EB1)
  [in7] -> M191/4(CT2)
  [in8] -> M191/5(F2)
  [in9] -> M191/6(E2)
  [in10] -> M191/7(MR2)
  [in11] -> M191/8(T2)
  [in12] -> M191/9(EB2)
  [in13] -> M191/10(CT3)
  [in17] -> M191/11(T3)
  [in18] -> M191/12(EB3)
  M191/1(LL1) -> Eval190/1(In1)
  M191/2(LL2) -> Eval190/2(In2)
  M191/3(LL3) -> Eval190/3(In3)
  Eval190/1(Out1) -> To Workspace190/1
  [in1] -> M192/1(CT1)
  [in5] -> M192/2(T1)
  [in6] -> M192/3(EB1)
  [in7] -> M192/4(CT2)
  [in8] -> M192/5(F2)
  [in9] -> M192/6(E2)
  [in10] -> M192/7(MR2)
  [in11] -> M192/8(T2)
  [in12] -> M192/9(EB2)
  [in13] -> M192/10(CT3)
  [in17] -> M192/11(T3)
  [in18] -> M192/12(EB3)
  M192/1(LL1) -> Eval191/1(In1)
  M192/2(LL2) -> Eval191/2(In2)
  M192/3(LL3) -> Eval191/3(In3)
  Eval191/1(Out1) -> To Workspace191/1
  [in1] -> M193/1(CT1)
  [in5] -> M193/2(T1)
  [in6] -> M193/3(EB1)
  [in7] -> M193/4(CT2)
  [in8] -> M193/5(F2)
  [in9] -> M193/6(E2)
  [in10] -> M193/7(MR2)
  [in11] -> M193/8(T2)
  [in12] -> M193/9(EB2)
  [in13] -> M193/10(CT3)
  [in17] -> M193/11(T3)
  [in18] -> M193/12(EB3)
  M193/1(LL1) -> Eval192/1(In1)
  M193/2(LL2) -> Eval192/2(In2)
  M193/3(LL3) -> Eval192/3(In3)
  Eval192/1(Out1) -> To Workspace192/1
  [in1] -> M194/1(CT1)
  [in5] -> M194/2(T1)
  [in6] -> M194/3(EB1)
  [in7] -> M194/4(CT2)
  [in8] -> M194/5(F2)
  [in9] -> M194/6(E2)
  [in10] -> M194/7(MR2)
  [in11] -> M194/8(T2)
  [in12] -> M194/9(EB2)
  [in13] -> M194/10(CT3)
  [in17] -> M194/11(T3)
  [in18] -> M194/12(EB3)
  M194/1(LL1) -> Eval193/1(In1)
  M194/2(LL2) -> Eval193/2(In2)
  M194/3(LL3) -> Eval193/3(In3)
  Eval193/1(Out1) -> To Workspace193/1
  [in1] -> M195/1(CT1)
  [in5] -> M195/2(T1)
  [in6] -> M195/3(EB1)
  [in7] -> M195/4(CT2)
  [in8] -> M195/5(F2)
  [in9] -> M195/6(E2)
  [in10] -> M195/7(MR2)
  [in11] -> M195/8(T2)
  [in12] -> M195/9(EB2)
  [in13] -> M195/10(CT3)
  [in17] -> M195/11(T3)
  [in18] -> M195/12(EB3)
  M195/1(LL1) -> Eval194/1(In1)
  M195/2(LL2) -> Eval194/2(In2)
  M195/3(LL3) -> Eval194/3(In3)
  Eval194/1(Out1) -> To Workspace194/1
  [in1] -> M196/1(CT1)
  [in5] -> M196/2(T1)
  [in6] -> M196/3(EB1)
  [in7] -> M196/4(CT2)
  [in8] -> M196/5(F2)
  [in9] -> M196/6(E2)
  [in10] -> M196/7(MR2)
  [in11] -> M196/8(T2)
  [in12] -> M196/9(EB2)
  [in13] -> M196/10(CT3)
  [in17] -> M196/11(T3)
  [in18] -> M196/12(EB3)
  M196/1(LL1) -> Eval195/1(In1)
  M196/2(LL2) -> Eval195/2(In2)
  M196/3(LL3) -> Eval195/3(In3)
  Eval195/1(Out1) -> To Workspace195/1
  [in1] -> M197/1(CT1)
  [in5] -> M197/2(T1)
  [in6] -> M197/3(EB1)
  [in7] -> M197/4(CT2)
  [in8] -> M197/5(F2)
  [in9] -> M197/6(E2)
  [in10] -> M197/7(MR2)
  [in11] -> M197/8(T2)
  [in12] -> M197/9(EB2)
  [in13] -> M197/10(CT3)
  [in17] -> M197/11(T3)
  [in18] -> M197/12(EB3)
  M197/1(LL1) -> Eval196/1(In1)
  M197/2(LL2) -> Eval196/2(In2)
  M197/3(LL3) -> Eval196/3(In3)
  Eval196/1(Out1) -> To Workspace196/1
  [in1] -> M198/1(CT1)
  [in5] -> M198/2(T1)
  [in6] -> M198/3(EB1)
  [in7] -> M198/4(CT2)
  [in8] -> M198/5(F2)
  [in9] -> M198/6(E2)
  [in10] -> M198/7(MR2)
  [in11] -> M198/8(T2)
  [in12] -> M198/9(EB2)
  [in13] -> M198/10(CT3)
  [in17] -> M198/11(T3)
  [in18] -> M198/12(EB3)
  M198/1(LL1) -> Eval197/1(In1)
  M198/2(LL2) -> Eval197/2(In2)
  M198/3(LL3) -> Eval197/3(In3)
  Eval197/1(Out1) -> To Workspace197/1
  [in1] -> M199/1(CT1)
  [in5] -> M199/2(T1)
  [in6] -> M199/3(EB1)
  [in7] -> M199/4(CT2)
  [in8] -> M199/5(F2)
  [in9] -> M199/6(E2)
  [in10] -> M199/7(MR2)
  [in11] -> M199/8(T2)
  [in12] -> M199/9(EB2)
  [in13] -> M199/10(CT3)
  [in17] -> M199/11(T3)
  [in18] -> M199/12(EB3)
  M199/1(LL1) -> Eval198/1(In1)
  M199/2(LL2) -> Eval198/2(In2)
  M199/3(LL3) -> Eval198/3(In3)
  Eval198/1(Out1) -> To Workspace198/1
  [in1] -> M221/1(CT1)
  [in5] -> M221/2(T1)
  [in6] -> M221/3(EB1)
  [in7] -> M221/4(CT2)
  [in8] -> M221/5(F2)
  [in9] -> M221/6(E2)
  [in10] -> M221/7(MR2)
  [in11] -> M221/8(T2)
  [in12] -> M221/9(EB2)
  [in13] -> M221/10(CT3)
  [in17] -> M221/11(T3)
  [in18] -> M221/12(EB3)
  M221/1(LL1) -> Eval220/1(In1)
  M221/2(LL2) -> Eval220/2(In2)
  M221/3(LL3) -> Eval220/3(In3)
  Eval220/1(Out1) -> To Workspace220/1
  [in1] -> M222/1(CT1)
  [in5] -> M222/2(T1)
  [in6] -> M222/3(EB1)
  [in7] -> M222/4(CT2)
  [in8] -> M222/5(F2)
  [in9] -> M222/6(E2)
  [in10] -> M222/7(MR2)
  [in11] -> M222/8(T2)
  [in12] -> M222/9(EB2)
  [in13] -> M222/10(CT3)
  [in17] -> M222/11(T3)
  [in18] -> M222/12(EB3)
  M222/1(LL1) -> Eval221/1(In1)
  M222/2(LL2) -> Eval221/2(In2)
  M222/3(LL3) -> Eval221/3(In3)
  Eval221/1(Out1) -> To Workspace221/1
  [in1] -> M223/1(CT1)
  [in5] -> M223/2(T1)
  [in6] -> M223/3(EB1)
  [in7] -> M223/4(CT2)
  [in8] -> M223/5(F2)
  [in9] -> M223/6(E2)
  [in10] -> M223/7(MR2)
  [in11] -> M223/8(T2)
  [in12] -> M223/9(EB2)
  [in13] -> M223/10(CT3)
  [in17] -> M223/11(T3)
  [in18] -> M223/12(EB3)
  M223/1(LL1) -> Eval222/1(In1)
  M223/2(LL2) -> Eval222/2(In2)
  M223/3(LL3) -> Eval222/3(In3)
  Eval222/1(Out1) -> To Workspace222/1
  [in1] -> M224/1(CT1)
  [in5] -> M224/2(T1)
  [in6] -> M224/3(EB1)
  [in7] -> M224/4(CT2)
  [in8] -> M224/5(F2)
  [in9] -> M224/6(E2)
  [in10] -> M224/7(MR2)
  [in11] -> M224/8(T2)
  [in12] -> M224/9(EB2)
  [in13] -> M224/10(CT3)
  [in17] -> M224/11(T3)
  [in18] -> M224/12(EB3)
  M224/1(LL1) -> Eval223/1(In1)
  M224/2(LL2) -> Eval223/2(In2)
  M224/3(LL3) -> Eval223/3(In3)
  Eval223/1(Out1) -> To Workspace223/1
  [in1] -> M225/1(CT1)
  [in5] -> M225/2(T1)
  [in6] -> M225/3(EB1)
  [in7] -> M225/4(CT2)
  [in8] -> M225/5(F2)
  [in9] -> M225/6(E2)
  [in10] -> M225/7(MR2)
  [in11] -> M225/8(T2)
  [in12] -> M225/9(EB2)
  [in13] -> M225/10(CT3)
  [in17] -> M225/11(T3)
  [in18] -> M225/12(EB3)
  M225/1(LL1) -> Eval224/1(In1)
  M225/2(LL2) -> Eval224/2(In2)
  M225/3(LL3) -> Eval224/3(In3)
  Eval224/1(Out1) -> To Workspace224/1
  [in1] -> M226/1(CT1)
  [in5] -> M226/2(T1)
  [in6] -> M226/3(EB1)
  [in7] -> M226/4(CT2)
  [in8] -> M226/5(F2)
  [in9] -> M226/6(E2)
  [in10] -> M226/7(MR2)
  [in11] -> M226/8(T2)
  [in12] -> M226/9(EB2)
  [in13] -> M226/10(CT3)
  [in17] -> M226/11(T3)
  [in18] -> M226/12(EB3)
  M226/1(LL1) -> Eval225/1(In1)
  M226/2(LL2) -> Eval225/2(In2)
  M226/3(LL3) -> Eval225/3(In3)
  Eval225/1(Out1) -> To Workspace225/1
  [in1] -> M227/1(CT1)
  [in5] -> M227/2(T1)
  [in6] -> M227/3(EB1)
  [in7] -> M227/4(CT2)
  [in8] -> M227/5(F2)
  [in9] -> M227/6(E2)
  [in10] -> M227/7(MR2)
  [in11] -> M227/8(T2)
  [in12] -> M227/9(EB2)
  [in13] -> M227/10(CT3)
  [in17] -> M227/11(T3)
  [in18] -> M227/12(EB3)
  M227/1(LL1) -> Eval226/1(In1)
  M227/2(LL2) -> Eval226/2(In2)
  M227/3(LL3) -> Eval226/3(In3)
  Eval226/1(Out1) -> To Workspace226/1
  [in1] -> M228/1(CT1)
  [in5] -> M228/2(T1)
  [in6] -> M228/3(EB1)
  [in7] -> M228/4(CT2)
  [in8] -> M228/5(F2)
  [in9] -> M228/6(E2)
  [in10] -> M228/7(MR2)
  [in11] -> M228/8(T2)
  [in12] -> M228/9(EB2)
  [in13] -> M228/10(CT3)
  [in17] -> M228/11(T3)
  [in18] -> M228/12(EB3)
  M228/1(LL1) -> Eval227/1(In1)
  M228/2(LL2) -> Eval227/2(In2)
  M228/3(LL3) -> Eval227/3(In3)
  Eval227/1(Out1) -> To Workspace227/1
  [in1] -> M229/1(CT1)
  [in5] -> M229/2(T1)
  [in6] -> M229/3(EB1)
  [in7] -> M229/4(CT2)
  [in8] -> M229/5(F2)
  [in9] -> M229/6(E2)
  [in10] -> M229/7(MR2)
  [in11] -> M229/8(T2)
  [in12] -> M229/9(EB2)
  [in13] -> M229/10(CT3)
  [in17] -> M229/11(T3)
  [in18] -> M229/12(EB3)
  M229/1(LL1) -> Eval228/1(In1)
  M229/2(LL2) -> Eval228/2(In2)
  M229/3(LL3) -> Eval228/3(In3)
  Eval228/1(Out1) -> To Workspace228/1
  [in1] -> M230/1(CT1)
  [in5] -> M230/2(T1)
  [in6] -> M230/3(EB1)
  [in7] -> M230/4(CT2)
  [in8] -> M230/5(F2)
  [in9] -> M230/6(E2)
  [in10] -> M230/7(MR2)
  [in11] -> M230/8(T2)
  [in12] -> M230/9(EB2)
  [in13] -> M230/10(CT3)
  [in17] -> M230/11(T3)
  [in18] -> M230/12(EB3)
  M230/1(LL1) -> Eval229/1(In1)
  M230/2(LL2) -> Eval229/2(In2)
  M230/3(LL3) -> Eval229/3(In3)
  Eval229/1(Out1) -> To Workspace229/1
  [in1] -> M231/1(CT1)
  [in5] -> M231/2(T1)
  [in6] -> M231/3(EB1)
  [in7] -> M231/4(CT2)
  [in8] -> M231/5(F2)
  [in9] -> M231/6(E2)
  [in10] -> M231/7(MR2)
  [in11] -> M231/8(T2)
  [in12] -> M231/9(EB2)
  [in13] -> M231/10(CT3)
  [in17] -> M231/11(T3)
  [in18] -> M231/12(EB3)
  M231/1(LL1) -> Eval230/1(In1)
  M231/2(LL2) -> Eval230/2(In2)
  M231/3(LL3) -> Eval230/3(In3)
  Eval230/1(Out1) -> To Workspace230/1
  [in1] -> M232/1(CT1)
  [in5] -> M232/2(T1)
  [in6] -> M232/3(EB1)
  [in7] -> M232/4(CT2)
  [in8] -> M232/5(F2)
  [in9] -> M232/6(E2)
  [in10] -> M232/7(MR2)
  [in11] -> M232/8(T2)
  [in12] -> M232/9(EB2)
  [in13] -> M232/10(CT3)
  [in17] -> M232/11(T3)
  [in18] -> M232/12(EB3)
  M232/1(LL1) -> Eval231/1(In1)
  M232/2(LL2) -> Eval231/2(In2)
  M232/3(LL3) -> Eval231/3(In3)
  Eval231/1(Out1) -> To Workspace231/1
  [in1] -> M233/1(CT1)
  [in5] -> M233/2(T1)
  [in6] -> M233/3(EB1)
  [in7] -> M233/4(CT2)
  [in8] -> M233/5(F2)
  [in9] -> M233/6(E2)
  [in10] -> M233/7(MR2)
  [in11] -> M233/8(T2)
  [in12] -> M233/9(EB2)
  [in13] -> M233/10(CT3)
  [in17] -> M233/11(T3)
  [in18] -> M233/12(EB3)
  M233/1(LL1) -> Eval232/1(In1)
  M233/2(LL2) -> Eval232/2(In2)
  M233/3(LL3) -> Eval232/3(In3)
  Eval232/1(Out1) -> To Workspace232/1
  [in1] -> M234/1(CT1)
  [in5] -> M234/2(T1)
  [in6] -> M234/3(EB1)
  [in7] -> M234/4(CT2)
  [in8] -> M234/5(F2)
  [in9] -> M234/6(E2)
  [in10] -> M234/7(MR2)
  [in11] -> M234/8(T2)
  [in12] -> M234/9(EB2)
  [in13] -> M234/10(CT3)
  [in17] -> M234/11(T3)
  [in18] -> M234/12(EB3)
  M234/1(LL1) -> Eval233/1(In1)
  M234/2(LL2) -> Eval233/2(In2)
  M234/3(LL3) -> Eval233/3(In3)
  Eval233/1(Out1) -> To Workspace233/1
  [in1] -> M235/1(CT1)
  [in5] -> M235/2(T1)
  [in6] -> M235/3(EB1)
  [in7] -> M235/4(CT2)
  [in8] -> M235/5(F2)
  [in9] -> M235/6(E2)
  [in10] -> M235/7(MR2)
  [in11] -> M235/8(T2)
  [in12] -> M235/9(EB2)
  [in13] -> M235/10(CT3)
  [in17] -> M235/11(T3)
  [in18] -> M235/12(EB3)
  M235/1(LL1) -> Eval234/1(In1)
  M235/2(LL2) -> Eval234/2(In2)
  M235/3(LL3) -> Eval234/3(In3)
  Eval234/1(Out1) -> To Workspace234/1
  [in1] -> M236/1(CT1)
  [in5] -> M236/2(T1)
  [in6] -> M236/3(EB1)
  [in7] -> M236/4(CT2)
  [in8] -> M236/5(F2)
  [in9] -> M236/6(E2)
  [in10] -> M236/7(MR2)
  [in11] -> M236/8(T2)
  [in12] -> M236/9(EB2)
  [in13] -> M236/10(CT3)
  [in17] -> M236/11(T3)
  [in18] -> M236/12(EB3)
  M236/1(LL1) -> Eval235/1(In1)
  M236/2(LL2) -> Eval235/2(In2)
  M236/3(LL3) -> Eval235/3(In3)
  Eval235/1(Out1) -> To Workspace235/1
  [in1] -> M237/1(CT1)
  [in5] -> M237/2(T1)
  [in6] -> M237/3(EB1)
  [in7] -> M237/4(CT2)
  [in8] -> M237/5(F2)
  [in9] -> M237/6(E2)
  [in10] -> M237/7(MR2)
  [in11] -> M237/8(T2)
  [in12] -> M237/9(EB2)
  [in13] -> M237/10(CT3)
  [in17] -> M237/11(T3)
  [in18] -> M237/12(EB3)
  M237/1(LL1) -> Eval236/1(In1)
  M237/2(LL2) -> Eval236/2(In2)
  M237/3(LL3) -> Eval236/3(In3)
  Eval236/1(Out1) -> To Workspace236/1
  [in1] -> M238/1(CT1)
  [in5] -> M238/2(T1)
  [in6] -> M238/3(EB1)
  [in7] -> M238/4(CT2)
  [in8] -> M238/5(F2)
  [in9] -> M238/6(E2)
  [in10] -> M238/7(MR2)
  [in11] -> M238/8(T2)
  [in12] -> M238/9(EB2)
  [in13] -> M238/10(CT3)
  [in17] -> M238/11(T3)
  [in18] -> M238/12(EB3)
  M238/1(LL1) -> Eval237/1(In1)
  M238/2(LL2) -> Eval237/2(In2)
  M238/3(LL3) -> Eval237/3(In3)
  Eval237/1(Out1) -> To Workspace237/1
  [in1] -> M239/1(CT1)
  [in5] -> M239/2(T1)
  [in6] -> M239/3(EB1)
  [in7] -> M239/4(CT2)
  [in8] -> M239/5(F2)
  [in9] -> M239/6(E2)
  [in10] -> M239/7(MR2)
  [in11] -> M239/8(T2)
  [in12] -> M239/9(EB2)
  [in13] -> M239/10(CT3)
  [in17] -> M239/11(T3)
  [in18] -> M239/12(EB3)
  M239/1(LL1) -> Eval238/1(In1)
  M239/2(LL2) -> Eval238/2(In2)
  M239/3(LL3) -> Eval238/3(In3)
  Eval238/1(Out1) -> To Workspace238/1
  [in1] -> M240/1(CT1)
  [in5] -> M240/2(T1)
  [in6] -> M240/3(EB1)
  [in7] -> M240/4(CT2)
  [in8] -> M240/5(F2)
  [in9] -> M240/6(E2)
  [in10] -> M240/7(MR2)
  [in11] -> M240/8(T2)
  [in12] -> M240/9(EB2)
  [in13] -> M240/10(CT3)
  [in17] -> M240/11(T3)
  [in18] -> M240/12(EB3)
  M240/1(LL1) -> Eval239/1(In1)
  M240/2(LL2) -> Eval239/2(In2)
  M240/3(LL3) -> Eval239/3(In3)
  Eval239/1(Out1) -> To Workspace239/1
  [in1] -> M241/1(CT1)
  [in5] -> M241/2(T1)
  [in6] -> M241/3(EB1)
  [in7] -> M241/4(CT2)
  [in8] -> M241/5(F2)
  [in9] -> M241/6(E2)
  [in10] -> M241/7(MR2)
  [in11] -> M241/8(T2)
  [in12] -> M241/9(EB2)
  [in13] -> M241/10(CT3)
  [in17] -> M241/11(T3)
  [in18] -> M241/12(EB3)
  M241/1(LL1) -> Eval240/1(In1)
  M241/2(LL2) -> Eval240/2(In2)
  M241/3(LL3) -> Eval240/3(In3)
  Eval240/1(Out1) -> To Workspace240/1
  [in1] -> M242/1(CT1)
  [in5] -> M242/2(T1)
  [in6] -> M242/3(EB1)
  [in7] -> M242/4(CT2)
  [in8] -> M242/5(F2)
  [in9] -> M242/6(E2)
  [in10] -> M242/7(MR2)
  [in11] -> M242/8(T2)
  [in12] -> M242/9(EB2)
  [in13] -> M242/10(CT3)
  [in17] -> M242/11(T3)
  [in18] -> M242/12(EB3)
  M242/1(LL1) -> Eval241/1(In1)
  M242/2(LL2) -> Eval241/2(In2)
  M242/3(LL3) -> Eval241/3(In3)
  Eval241/1(Out1) -> To Workspace241/1
  [in1] -> M243/1(CT1)
  [in5] -> M243/2(T1)
  [in6] -> M243/3(EB1)
  [in7] -> M243/4(CT2)
  [in8] -> M243/5(F2)
  [in9] -> M243/6(E2)
  [in10] -> M243/7(MR2)
  [in11] -> M243/8(T2)
  [in12] -> M243/9(EB2)
  [in13] -> M243/10(CT3)
  [in17] -> M243/11(T3)
  [in18] -> M243/12(EB3)
  M243/1(LL1) -> Eval242/1(In1)
  M243/2(LL2) -> Eval242/2(In2)
  M243/3(LL3) -> Eval242/3(In3)
  Eval242/1(Out1) -> To Workspace242/1
  [in1] -> M244/1(CT1)
  [in5] -> M244/2(T1)
  [in6] -> M244/3(EB1)
  [in7] -> M244/4(CT2)
  [in8] -> M244/5(F2)
  [in9] -> M244/6(E2)
  [in10] -> M244/7(MR2)
  [in11] -> M244/8(T2)
  [in12] -> M244/9(EB2)
  [in13] -> M244/10(CT3)
  [in17] -> M244/11(T3)
  [in18] -> M244/12(EB3)
  M244/1(LL1) -> Eval243/1(In1)
  M244/2(LL2) -> Eval243/2(In2)
  M244/3(LL3) -> Eval243/3(In3)
  Eval243/1(Out1) -> To Workspace243/1
  [in1] -> M245/1(CT1)
  [in5] -> M245/2(T1)
  [in6] -> M245/3(EB1)
  [in7] -> M245/4(CT2)
  [in8] -> M245/5(F2)
  [in9] -> M245/6(E2)
  [in10] -> M245/7(MR2)
  [in11] -> M245/8(T2)
  [in12] -> M245/9(EB2)
  [in13] -> M245/10(CT3)
  [in17] -> M245/11(T3)
  [in18] -> M245/12(EB3)
  M245/1(LL1) -> Eval244/1(In1)
  M245/2(LL2) -> Eval244/2(In2)
  M245/3(LL3) -> Eval244/3(In3)
  Eval244/1(Out1) -> To Workspace244/1
  [in1] -> M246/1(CT1)
  [in5] -> M246/2(T1)
  [in6] -> M246/3(EB1)
  [in7] -> M246/4(CT2)
  [in8] -> M246/5(F2)
  [in9] -> M246/6(E2)
  [in10] -> M246/7(MR2)
  [in11] -> M246/8(T2)
  [in12] -> M246/9(EB2)
  [in13] -> M246/10(CT3)
  [in17] -> M246/11(T3)
  [in18] -> M246/12(EB3)
  M246/1(LL1) -> Eval245/1(In1)
  M246/2(LL2) -> Eval245/2(In2)
  M246/3(LL3) -> Eval245/3(In3)
  Eval245/1(Out1) -> To Workspace245/1
  Inputs/1(CT1) -> dtc_CT1/1
  dtc_CT1/1 -> CPSUT/1(CT1), [in1]
  Inputs/2(T1) -> dtc_T1/1
  dtc_T1/1 -> CPSUT/2(T1), [in5]
  Inputs/3(EB1) -> dtc_EB1/1
  dtc_EB1/1 -> CPSUT/3(EB1), [in6]
  Inputs/4(CT2) -> dtc_CT2/1
  dtc_CT2/1 -> CPSUT/4(CT2), [in7]
  Inputs/5(F2) -> dtc_F2/1
  dtc_F2/1 -> CPSUT/5(F2), [in8]
  Inputs/6(E2) -> dtc_E2/1
  dtc_E2/1 -> CPSUT/6(E2), [in9]
  Inputs/7(MR2) -> dtc_MR2/1
  dtc_MR2/1 -> CPSUT/7(MR2), [in10]
  Inputs/8(T2) -> dtc_T2/1
  dtc_T2/1 -> CPSUT/8(T2), [in11]
  Inputs/9(EB2) -> dtc_EB2/1
  dtc_EB2/1 -> CPSUT/9(EB2), [in12]
  Inputs/10(CT3) -> dtc_CT3/1
  dtc_CT3/1 -> CPSUT/10(CT3), [in13]
  Inputs/11(T3) -> dtc_T3/1
  dtc_T3/1 -> CPSUT/11(T3), [in17]
  Inputs/12(EB3) -> dtc_EB3/1
  dtc_EB3/1 -> CPSUT/12(EB3), [in18]
